simulink model "HMC"  (R2026a)
settings: Solver=ode1  StopTime=inf  FixedStep=0.0001
PreLoadFcn:
  | %load('C:\Users\bme_master\Desktop\mot\mot_6_deneme.mat')
  | 
  | 
  | %load('C:\Users\bme_master\Desktop\mot\PRE_G''s.mat')
PostLoadFcn:
  | , if any(exist('dsrtsu_mdlpostloadfcn', 'file') ~= 0), dsrtsu_mdlpostloadfcn('Execute', bdroot); end,
InitFcn:
  | %motor_control_init_m
  | %clear all
  | %close all
  | %clc
  | b=1e-8
  | StepSize = 1e-4;
  | N=1e-17;
  | 
  | VLV_0 =0;%120; %120
  | VA_0 = 0;%300; %300
  | VRV_0 = 0;%130;
  | VP_0 = 0;%500;
  | VLA_0 = 0;%20;
  | VV_0=5000;
  | VRA_0=0;
  | 
  | 
  | QLV_0 = 0;
  | QLA_0 = 0;
  | QP_0 = 0;
  | 
  | bh = 0;
  | th =0;
  | 
  | X_0 = [VLV_0 VA_0 VV_0 VP_0  VLA_0  VRA_0 VRV_0];
  | 
  | 
  | V0 = 10;
  | 
  | K1=.0004;%0.0001
  | K2=0.0009;%0.0009
  | KA=1;%1
  | C1=0.000000003;%0.0000003
  | lambda=6000;%3000
  | X_00 = [VLV_0 VA_0 VV_0 VRV_0];
  | 
  | r2 = 0.05/2;
  | A2 = pi*r2^2;
  | h2 = 0.63;
  | V2 = A2*h2;
  | 
  | 
  | r3 = 0.05/2;
  | A3 = pi*r3^2;
  | h3 = 0.63;
  | V3 = A3*h3;
  | 
  | 
  | rho = 997;
  | gg = 9.81;
  | %
  | init_min=0;
  | init_max=0;
  | %
  | PWM_Period =  StepSize;
  | PWM_Period_g1 = PWM_Period;
  | PWM_Period_g2 =PWM_Period;
  | PWM_Period_g3 = PWM_Period;
  | PWM_Period_g4 = PWM_Period;
  | PWM_Period_g5 = PWM_Period;
  | PWM_Period_P2_escape = PWM_Period;
  | PWM_Period_P3_escape = PWM_Period;
  | filter_c=100;
  | dt = StepSize;
  | dt_k = dt;
  | rho_g=1.537408456055604
  | Pvac = 0;
  | P1refmmHg = 1600;
  | P2refmmHg = 30;
  | 
  | 
  | P2_ref_freq = 1;
  | P2_ref_bias = 50;
  | P2_ref_amp = 0;
  | P2_ref_shift = 0;
  | Kp = 1;
  | Ki =1;
  | Kd=1;
  | 
  | 
  | P3_ref_freq = 1;
  | P3_ref_bias = 30;
  | P3_ref_amp = 0;
  | P3_ref_shift = 0;
  | 
  | Q_Sys_std = 1;
  | R_Meas_std = 1;
  | kalmanP_in= [133.32*[100 1 10 10 1]]';
  | kalmanQ_in = [1e-3 1e-3]';
  | y_kalman_ini = [133.32*[100 1 10 10 1] 1e-3 1e-3 1e-3]';
  | P_kalman_ini = R_Meas_std^2*eye(8);
  | %P_kalman_ini = R_Meas_std^2*eye(8);
  | %P_kalman_in1 = R_Meas_std^2*eye(8);
  | 
  | 
  | w_gp_0 = 1e-3;
  | i_gp_0 = 1e-3;
  | w_vad_0 = 1e-3;
  | i_vad_0 = 1e-3;
  | 
  | 
  | 
  | 
  | 
  | % e_min = 0.075;
  | % %e_max = 3;
  | % e_max_ill = 1.5; PA_0 = 85;
  | % tau_RA = 1.8;  tau_RV = 3;% 2.3762;
  | % V_total = 5500; V0_la = 70; V0_lv = 120; V0 = 10;
  | % RA = 1.2; Ra = 0.0005;
  | % Rm = 0.0003; Rv = 0.005;
  | % R = [RA Ra Rm Rv];
  | % g = [1/RA 1/Ra 1/Rm 1/Rv];
  | %
  | % CA = tau_RA/RA; CV = tau_RV/Rv;
  | %
  | % V0_aortic = PA_0*CA;
  | % PLV_0 = (V0_lv - V0)*e_min;
  | % CLA = V0_la/PLV_0;
  | % C = [CA CV CLA];
  | % e = [1/CA 1/CV 1/CLA];
  | %
  | % V0_venous = V_total - (V0_aortic + V0_la + V0_lv);
  | % PLA_0 = PLV_0;
  | % PV_0 = V0_venous/CV;
  | 
  | 
  | 
  | 
  | 
  | 
  | 
  | 
  | % stepsize = 1e-4;
  | 
  | % SS=1;
  | 
  | 
  | 
  | 
  | 
  | %global RFa RFp
  | %RFa = 1;
  | %RFmv = 1;
  | 
  | 
  | 
  | 
  | 
  | %L_AV =  0.000232;
  | %L_mv =  0.0001;
  | %L_P =  0.000128;
  | a=0;
  | 
  | 
  | 
  | 
  | 
  | %L= [L_mv];
  | 
  | 
  | 
  | 
  | 
  | % gLV =42;%25;
  | % gA = 0.9225;%0.75;  %0.8;%0.725; %1.11;
  | % gV = 70;%10000;
  | % gRV =210;
  | % gP =5;%15 %10;
  | % gLA = 1000; %1000;
  | %
  | %
  | % G = [gLV gA gV gRV gP gLA];
  | %
  | %
  | % eA =0.5225;%0.725;%1; %0.925;%0.83; %0.65;%0.95;
  | % eV =0.002425;%0.00245;%0.00125;
  | % eP =0.1; %0.01%0.1;
  | % eLA =0.1025;%0.1105%0.1175;%0.15; % 0.15;
  | %
  | %
  | % E = [eA eV eP eLA];
  | %
  | %
  | % ZZ = 0.75;
  | % PP = 0.95;
  | %
  | % V_T = 5000;
  | % VLV_0 =105;%120; %120
  | % VA_0 = 160;%300; %300
  | % VRV_0 = 110;%130;
  | % VP_0 = 200;%500;
  | % VLA_0 = 105;%20;
  | % VV_0=0;
  | % QLV_0 = 0;
  | % QLA_0 = 0;
  | % QP_0 = 0;
  | %
  | % X_0 = [VLV_0 VA_0 VRV_0 VP_0 VLA_0];
  | % %BF_0 = [0 0 0];
  | %
  | %
  | % V0 = 10;
  | 
  | 
  | %Delay = 0.85;
  | 
  | 
  | 
  | 
  | 
  | %%CVS PARAMETERS NEW
  | 
  | 
  | stepsize = 1e-4;
  | 
  | 
  | SS=0.8;
undefined symbols (not defined in the file or in its folder): Continuous, DiscIntNeverNeededParam, Time
libraries: powerlib_meascontrol x19, simulink x15, rti1202lib_adc_class1 x11, cstblocks x10, rti1202lib_dio_class1 x8, dspstat3 x3, rti1202lib_dac_class1 x1, dspswit3 x1, ctrlSharedLib x1, slpidlib x1, dsparch4 x1
(part 1 of 5)
Description:
  | Standard RTI1202 template.
  | Supported MATLAB version:  R2019a.
settings Model: Tag=RTI1202  DSRTSU_INTERNAL_RTI_VER=540  DSRTSU_INTERNAL_RTI_TYPE=rti1202  RTICANMMDATA=struct('GeneralSetupData',struct('modelroot','C:\Users\bme_master\Desktop\dSpaceEncoder','generalsettings',struct('filesettings',struct('destfolder',struct('Name','RTICANMM_FILES','Check',1),'buildfolder',struct('Name','.','Check',1),'AbsDestfolder',struct('Name','C:\Users\bme_master\Desktop\dSpaceEncoder\RTICANMM_FILES'),'AbsBuildfolder',struct('Name','C:\Users\bme_master\Desktop\dSpaceEncoder'))),'options',struct('addpaths',1,'rmpaths',1,'addtrcexclusion',logical(1),'cannavigator',struct('checkmonitoring',0),'show_usrtrc',0,'use_usrtrc',0),'advanced',struct('options',ones(1,100)),'MPSetup',{{}},'RTI',struct('Type','RTI1202','Ver','7.12','Date','02-May-2019'),'modelname','HMC','block','HMC'))  DSRTSU_INTERNAL_RTIFPGA=130  SimulationMode=accelerator  Creator=bme_master  LastModifiedBy=ehd
settings OptimizationCC: OptimizeBlockIOStorage=off  BufferReuse=off  GlobalBufferReuse=off  ExpressionFolding=off  LocalBlockOutputs=off  OptimizeDataStoreBuffers=off  BusAssignmentInplaceUpdate=off
settings HardwareCC: ProdLargestAtomicInteger=Integer  ProdEndianess=BigEndian  ProdHWDeviceType=Custom Processor->Custom  TargetIntDivRoundTo=Zero  TargetEndianess=BigEndian  TargetHWDeviceType=Custom Processor->Custom
settings RTWCC: SystemTargetFile=rti1202.tlc  MakeCommand=make_rti  TemplateMakefile=rti1202.tmf  Description=dSPACE DS1202 Hardware Platform
settings STFCustomTargetCC: SystemTargetFile=rti1202.tlc  MultiwordLength=2048.0  ParMdlRefBuildCompliant=on  GRTInterface=off  InitialSimState=RUN  ExecutionMode=real-time  ExecutionModeNonUI=RTSIM  TaskModeNonUI=LOW_JITTER  TaskMode=Low jitter, low latency tasks  AssertionMode=OFF  TimeScaleFactorNonUI=OPTION_DISABLED  TimeScaleFactor=1.0  EnableRealTimeTesting=on  EnableRealTimeTestingNonUI=ON  LoadAfterBuild=off  CCompilerOptimizationOptsPopup_=Default  CCompilerOptimizationOptsNonUI=USE_DEFAULT  AllowReservedHostServiceNums=off  BoardName=ds1202  RTICfgSetVer=540.0  LoadToFlash=off  TRCGenerateLabels=off  LoadApplNonUI=OFF  PlatformSelectionPopup=Platform Name  TRCGenerateVirtualBlocks=off  BoardNameNonUI=ds1202  NetworkClientNonUI=OPTION_DISABLED  TRCOnlyGlobals=off  TRCGenerateStates=off  TRCGenerateDerivatives=off  TRCGenerateParamValues=off  TRCIsOmitVdOn=off
settings GRTTargetCC: CompOptLevelCompliant=off  ConcurrentExecutionCompliant=off  CombineOutputUpdateFcns=off  MatFileLogging=off  CPPClassGenCompliant=off
settings ConfigComp: CovMetricSettings=dswe
settings SimscapeCC: SimscapeLogType=none  SimscapeNominalValues="[{\"value\":\"1\",\"unit\":\"A\"},{\"value\":\"1\",\"unit\":\"bar\"},{\"value\":\"1\",\"unit\":\"cm^2\"},{\"value\":\"1\",\"unit\":\"cm^3/s\"},{\"value\":\"1\",\"unit\":\"kJ/kg\"},{\"value\":\"1\",\"unit\":\"kW\"},{\"value\":\"1\",\"unit\":\"l\"},{\"value\":\"1\",\"unit\":\"N\"},{\"value\":\"1\",\"unit\":\"N*m\"},{\"value\":\"1\",\"unit\":\"V\"}]"  SimscapeLogDecimation=1  SimscapeLogDataHistory=5000

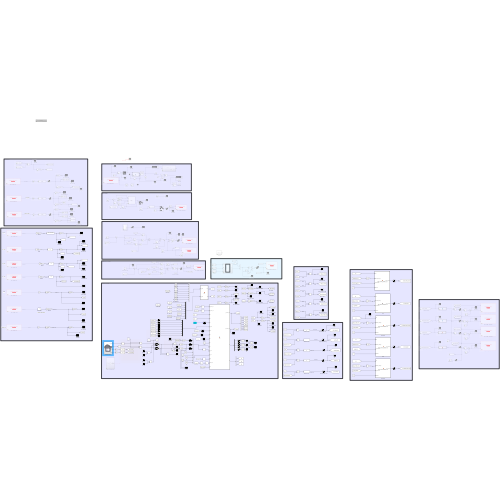
[thumbnail: Simulink's stored preview of the top-level diagram]
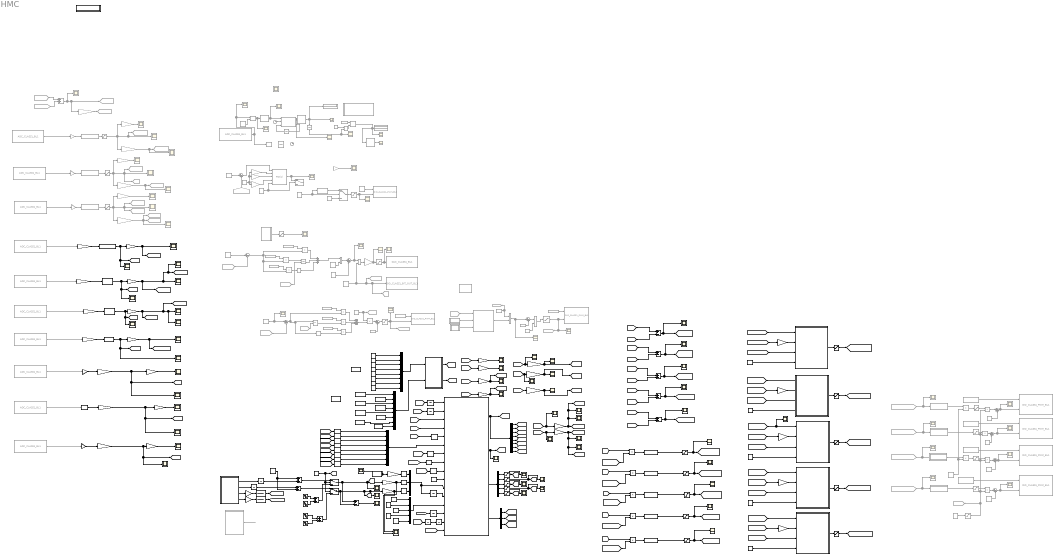
== system HMC ==
  note: ITM Controller
  note: Valve PWM
  note: Flow Sensors
  note: LV_total
  note: DTM LVAD contoller
  note: Ao_pne
  note: Small Pump Controller
  note: GP CONTROLLER
  note: -1 to 0 Bar Conversion
  note: Ao_total
  note: Between Tanks
  note: Comp
  note: Air Flows
  note: Valve Currents
  note: LV_pne
  note: Pressure Differences
  note: Pump Out
  note: Lyapunov controller
  note: Reduction_tank
  ADC_CLASS1_BL1 : rti1202lib_adc_class1/ADC_CLASS1_BL1  Commented=on  DSProperties=struct('RTI',struct('Version',uint32(1),'BlockType',struct('isSLSource',uint8(1),'isSLSink',uint8(1),'isHWSource',uint8(0),'isHWSink',uint8(1),'isSetup',uint8(0),'isInline',uint8(1),'isNonInline',uint8(0),'isInterrupt',uint8(0),'isChannelwise',uint8(1)),'IOBoardType',{{'DS120X','STD','ADCC1'}},'UnitType','ADC','Identifier','ADC','DialogType','ML','BlockSet','NONE','SlaveProcessor','NONE'))  RTIBlockInterface=struct('InputPortsActive',0,'InputPortsWidth',int32(1),'InputPortsDataType',{{'SS_BOOLEAN'}},'InputPortsName',{{'Continue'}},'OutputPortsActive',[1 0],'OutputPortsWidth',int32([1 1]),'OutputPortsDataType',{{'SS_DOUBLE','SS_INT16'}},'OutputPortsName',{{'ADC','Status'}},'DialogFcn','rti120xstdadcc1adcgui','SampleTime',{{-1}},'InitLevel',3,'IconTransparency','on','BlockDisplay',{{['ADC CL1\nChannel: 10'],'center'}},'BlockName',struct('Token',{{'ADC_CLASS1_BL1'}}))  RTIBlockParameters=struct('ReadMode',{{1,'OFF',[1 2]}},'ChannelNo',{{10,'OFF',[]}},'ConversionMode',{{1,'OFF',[1 2]}},'TriggerSource',{{1,'OFF',[1 2]}},'TriggerLineIn',{{1,'OFF',[1 16]}},'SampleMode',{{1,'OFF',[1 2]}},'BurstTriggerSource',{{1,'OFF',[1 2]}},'BurstTriggerLine',{{1,'OFF',[1 16]}},'ConvTriggerSource',{{3,'OFF',[1 3]}},'ConvTriggerLine',{{1,'OFF',[1 16]}},'ConvPeriod',{{'100e-6','OFF',[1e-6 1.34]}},'ConvPeriodCheck',{{0,'OFF',[]}},'BurstSize',{{'10','OFF',[]}},'BurstSizeCheck',{{0,'OFF',[]}},'DataSetOffset',{{'0','OFF',[]}},'DataSetOffsetCheck',{{0,'OFF',[]}},'DataSetLength',{{'1','OFF',[]}},'DataSetLengthCheck',{{0,'OFF',[]}},'EnableTriggerEvent',{{0,'OFF',[0 1]}},'TriggerMode',{{2,'OFF',[1 3]}},'TriggerLineOut',{{1,'OFF',[1 16]}},'ADCSWStartEnable',{{0,'OFF',[0 1]}},'SampleTime',{{'-1','OFF',[-1 inf]}},'SampleTimeCheck',{{1,'OFF',[]}},'StatusPortEnable',{{0,'OFF',[0 1]}},'TLCFileName',{{'rti120xadc_c1_adc','OFF',[]}})  RTISFcnParameters=struct('ReadMode','int16','ChannelNo','int16','ConversionMode','int16','TriggerSource','int16','TriggerLineIn','int16','SampleMode','int16','BurstTriggerSource','int16','BurstTriggerLine','int16','ConvTriggerSource','int16','ConvTriggerLine','int16','ConvPeriod','double','BurstSize','int16','DataSetOffset','int16','DataSetLength','int16','EnableTriggerEvent','int16','TriggerMode','int16','TriggerLineOut','int16','ADCSWStartEnable','int16','SampleTime','double','StatusPortEnable','int16','TLCFileName','char')  RTIBlockParaDefault=struct('ReadMode',1,'ChannelNo',1,'ConversionMode',1,'TriggerSource',1,'TriggerLineIn',1,'SampleMode',1,'BurstTriggerSource',1,'BurstTriggerLine',1,'ConvTriggerSource',3,'ConvTriggerLine',1,'ConvPeriod',0.0001,'ConvPeriodCheck',0,'BurstSize',10,'BurstSizeCheck',0,'DataSetOffset',0,'DataSetOffsetCheck',0,'DataSetLength',1,'DataSetLengthCheck',0,'EnableTriggerEvent',0,'TriggerMode',2,'TriggerLineOut',1,'ADCSWStartEnable',0,'SampleTime',-1,'SampleTimeCheck',1,'StatusPortEnable',0,'TLCFileName','rti120xadc_c1_adc')
  ADC_CLASS1_BL11 : rti1202lib_adc_class1/ADC_CLASS1_BL1  Commented=on  DSProperties=struct('RTI',struct('Version',uint32(1),'BlockType',struct('isSLSource',uint8(1),'isSLSink',uint8(1),'isHWSource',uint8(0),'isHWSink',uint8(1),'isSetup',uint8(0),'isInline',uint8(1),'isNonInline',uint8(0),'isInterrupt',uint8(0),'isChannelwise',uint8(1)),'IOBoardType',{{'DS120X','STD','ADCC1'}},'UnitType','ADC','Identifier','ADC','DialogType','ML','BlockSet','NONE','SlaveProcessor','NONE'))  RTIBlockInterface=struct('InputPortsActive',0,'InputPortsWidth',int32(1),'InputPortsDataType',{{'SS_BOOLEAN'}},'InputPortsName',{{'Continue'}},'OutputPortsActive',[1 0],'OutputPortsWidth',int32([1 1]),'OutputPortsDataType',{{'SS_DOUBLE','SS_INT16'}},'OutputPortsName',{{'ADC','Status'}},'DialogFcn','rti120xstdadcc1adcgui','SampleTime',{{-1}},'InitLevel',3,'IconTransparency','on','BlockDisplay',{{['ADC CL1\nChannel: 4'],'center'}},'BlockName',struct('Token',{{'ADC_CLASS1_BL1'}}))  RTIBlockParameters=struct('ReadMode',{{1,'OFF',[1 2]}},'ChannelNo',{{4,'OFF',[]}},'ConversionMode',{{1,'OFF',[1 2]}},'TriggerSource',{{1,'OFF',[1 2]}},'TriggerLineIn',{{1,'OFF',[1 16]}},'SampleMode',{{1,'OFF',[1 2]}},'BurstTriggerSource',{{1,'OFF',[1 2]}},'BurstTriggerLine',{{1,'OFF',[1 16]}},'ConvTriggerSource',{{3,'OFF',[1 3]}},'ConvTriggerLine',{{1,'OFF',[1 16]}},'ConvPeriod',{{'100e-6','OFF',[1e-6 1.34]}},'ConvPeriodCheck',{{0,'OFF',[]}},'BurstSize',{{'10','OFF',[]}},'BurstSizeCheck',{{0,'OFF',[]}},'DataSetOffset',{{'0','OFF',[]}},'DataSetOffsetCheck',{{0,'OFF',[]}},'DataSetLength',{{'1','OFF',[]}},'DataSetLengthCheck',{{0,'OFF',[]}},'EnableTriggerEvent',{{0,'OFF',[0 1]}},'TriggerMode',{{2,'OFF',[1 3]}},'TriggerLineOut',{{1,'OFF',[1 16]}},'ADCSWStartEnable',{{0,'OFF',[0 1]}},'SampleTime',{{'-1','OFF',[-1 inf]}},'SampleTimeCheck',{{1,'OFF',[]}},'StatusPortEnable',{{0,'OFF',[0 1]}},'TLCFileName',{{'rti120xadc_c1_adc','OFF',[]}})  RTISFcnParameters=struct('ReadMode','int16','ChannelNo','int16','ConversionMode','int16','TriggerSource','int16','TriggerLineIn','int16','SampleMode','int16','BurstTriggerSource','int16','BurstTriggerLine','int16','ConvTriggerSource','int16','ConvTriggerLine','int16','ConvPeriod','double','BurstSize','int16','DataSetOffset','int16','DataSetLength','int16','EnableTriggerEvent','int16','TriggerMode','int16','TriggerLineOut','int16','ADCSWStartEnable','int16','SampleTime','double','StatusPortEnable','int16','TLCFileName','char')  RTIBlockParaDefault=struct('ReadMode',1,'ChannelNo',1,'ConversionMode',1,'TriggerSource',1,'TriggerLineIn',1,'SampleMode',1,'BurstTriggerSource',1,'BurstTriggerLine',1,'ConvTriggerSource',3,'ConvTriggerLine',1,'ConvPeriod',0.0001,'ConvPeriodCheck',0,'BurstSize',10,'BurstSizeCheck',0,'DataSetOffset',0,'DataSetOffsetCheck',0,'DataSetLength',1,'DataSetLengthCheck',0,'EnableTriggerEvent',0,'TriggerMode',2,'TriggerLineOut',1,'ADCSWStartEnable',0,'SampleTime',-1,'SampleTimeCheck',1,'StatusPortEnable',0,'TLCFileName','rti120xadc_c1_adc')
  ADC_CLASS1_BL12 : rti1202lib_adc_class1/ADC_CLASS1_BL1  Commented=on  DSProperties=struct('RTI',struct('Version',uint32(1),'BlockType',struct('isSLSource',uint8(1),'isSLSink',uint8(1),'isHWSource',uint8(0),'isHWSink',uint8(1),'isSetup',uint8(0),'isInline',uint8(1),'isNonInline',uint8(0),'isInterrupt',uint8(0),'isChannelwise',uint8(1)),'IOBoardType',{{'DS120X','STD','ADCC1'}},'UnitType','ADC','Identifier','ADC','DialogType','ML','BlockSet','NONE','SlaveProcessor','NONE'))  RTIBlockInterface=struct('InputPortsActive',0,'InputPortsWidth',int32(1),'InputPortsDataType',{{'SS_BOOLEAN'}},'InputPortsName',{{'Continue'}},'OutputPortsActive',[1 0],'OutputPortsWidth',int32([1 1]),'OutputPortsDataType',{{'SS_DOUBLE','SS_INT16'}},'OutputPortsName',{{'ADC','Status'}},'DialogFcn','rti120xstdadcc1adcgui','SampleTime',{{-1}},'InitLevel',3,'IconTransparency','on','BlockDisplay',{{['ADC CL1\nChannel: 6'],'center'}},'BlockName',struct('Token',{{'ADC_CLASS1_BL1'}}))  RTIBlockParameters=struct('ReadMode',{{1,'OFF',[1 2]}},'ChannelNo',{{6,'OFF',[]}},'ConversionMode',{{1,'OFF',[1 2]}},'TriggerSource',{{1,'OFF',[1 2]}},'TriggerLineIn',{{1,'OFF',[1 16]}},'SampleMode',{{1,'OFF',[1 2]}},'BurstTriggerSource',{{1,'OFF',[1 2]}},'BurstTriggerLine',{{1,'OFF',[1 16]}},'ConvTriggerSource',{{3,'OFF',[1 3]}},'ConvTriggerLine',{{1,'OFF',[1 16]}},'ConvPeriod',{{'100e-6','OFF',[1e-6 1.34]}},'ConvPeriodCheck',{{0,'OFF',[]}},'BurstSize',{{'10','OFF',[]}},'BurstSizeCheck',{{0,'OFF',[]}},'DataSetOffset',{{'0','OFF',[]}},'DataSetOffsetCheck',{{0,'OFF',[]}},'DataSetLength',{{'1','OFF',[]}},'DataSetLengthCheck',{{0,'OFF',[]}},'EnableTriggerEvent',{{0,'OFF',[0 1]}},'TriggerMode',{{2,'OFF',[1 3]}},'TriggerLineOut',{{1,'OFF',[1 16]}},'ADCSWStartEnable',{{0,'OFF',[0 1]}},'SampleTime',{{'-1','OFF',[-1 inf]}},'SampleTimeCheck',{{1,'OFF',[]}},'StatusPortEnable',{{0,'OFF',[0 1]}},'TLCFileName',{{'rti120xadc_c1_adc','OFF',[]}})  RTISFcnParameters=struct('ReadMode','int16','ChannelNo','int16','ConversionMode','int16','TriggerSource','int16','TriggerLineIn','int16','SampleMode','int16','BurstTriggerSource','int16','BurstTriggerLine','int16','ConvTriggerSource','int16','ConvTriggerLine','int16','ConvPeriod','double','BurstSize','int16','DataSetOffset','int16','DataSetLength','int16','EnableTriggerEvent','int16','TriggerMode','int16','TriggerLineOut','int16','ADCSWStartEnable','int16','SampleTime','double','StatusPortEnable','int16','TLCFileName','char')  RTIBlockParaDefault=struct('ReadMode',1,'ChannelNo',1,'ConversionMode',1,'TriggerSource',1,'TriggerLineIn',1,'SampleMode',1,'BurstTriggerSource',1,'BurstTriggerLine',1,'ConvTriggerSource',3,'ConvTriggerLine',1,'ConvPeriod',0.0001,'ConvPeriodCheck',0,'BurstSize',10,'BurstSizeCheck',0,'DataSetOffset',0,'DataSetOffsetCheck',0,'DataSetLength',1,'DataSetLengthCheck',0,'EnableTriggerEvent',0,'TriggerMode',2,'TriggerLineOut',1,'ADCSWStartEnable',0,'SampleTime',-1,'SampleTimeCheck',1,'StatusPortEnable',0,'TLCFileName','rti120xadc_c1_adc')
  ADC_CLASS1_BL13 : rti1202lib_adc_class1/ADC_CLASS1_BL1  Commented=on  DSProperties=struct('RTI',struct('Version',uint32(1),'BlockType',struct('isSLSource',uint8(1),'isSLSink',uint8(1),'isHWSource',uint8(0),'isHWSink',uint8(1),'isSetup',uint8(0),'isInline',uint8(1),'isNonInline',uint8(0),'isInterrupt',uint8(0),'isChannelwise',uint8(1)),'IOBoardType',{{'DS120X','STD','ADCC1'}},'UnitType','ADC','Identifier','ADC','DialogType','ML','BlockSet','NONE','SlaveProcessor','NONE'))  RTIBlockInterface=struct('InputPortsActive',0,'InputPortsWidth',int32(1),'InputPortsDataType',{{'SS_BOOLEAN'}},'InputPortsName',{{'Continue'}},'OutputPortsActive',[1 0],'OutputPortsWidth',int32([1 1]),'OutputPortsDataType',{{'SS_DOUBLE','SS_INT16'}},'OutputPortsName',{{'ADC','Status'}},'DialogFcn','rti120xstdadcc1adcgui','SampleTime',{{-1}},'InitLevel',3,'IconTransparency','on','BlockDisplay',{{['ADC CL1\nChannel: 11'],'center'}},'BlockName',struct('Token',{{'ADC_CLASS1_BL1'}}))  RTIBlockParameters=struct('ReadMode',{{1,'OFF',[1 2]}},'ChannelNo',{{11,'OFF',[]}},'ConversionMode',{{1,'OFF',[1 2]}},'TriggerSource',{{1,'OFF',[1 2]}},'TriggerLineIn',{{1,'OFF',[1 16]}},'SampleMode',{{1,'OFF',[1 2]}},'BurstTriggerSource',{{1,'OFF',[1 2]}},'BurstTriggerLine',{{1,'OFF',[1 16]}},'ConvTriggerSource',{{3,'OFF',[1 3]}},'ConvTriggerLine',{{1,'OFF',[1 16]}},'ConvPeriod',{{'100e-6','OFF',[1e-6 1.34]}},'ConvPeriodCheck',{{0,'OFF',[]}},'BurstSize',{{'10','OFF',[]}},'BurstSizeCheck',{{0,'OFF',[]}},'DataSetOffset',{{'0','OFF',[]}},'DataSetOffsetCheck',{{0,'OFF',[]}},'DataSetLength',{{'1','OFF',[]}},'DataSetLengthCheck',{{0,'OFF',[]}},'EnableTriggerEvent',{{0,'OFF',[0 1]}},'TriggerMode',{{2,'OFF',[1 3]}},'TriggerLineOut',{{1,'OFF',[1 16]}},'ADCSWStartEnable',{{0,'OFF',[0 1]}},'SampleTime',{{'-1','OFF',[-1 inf]}},'SampleTimeCheck',{{1,'OFF',[]}},'StatusPortEnable',{{0,'OFF',[0 1]}},'TLCFileName',{{'rti120xadc_c1_adc','OFF',[]}})  RTISFcnParameters=struct('ReadMode','int16','ChannelNo','int16','ConversionMode','int16','TriggerSource','int16','TriggerLineIn','int16','SampleMode','int16','BurstTriggerSource','int16','BurstTriggerLine','int16','ConvTriggerSource','int16','ConvTriggerLine','int16','ConvPeriod','double','BurstSize','int16','DataSetOffset','int16','DataSetLength','int16','EnableTriggerEvent','int16','TriggerMode','int16','TriggerLineOut','int16','ADCSWStartEnable','int16','SampleTime','double','StatusPortEnable','int16','TLCFileName','char')  RTIBlockParaDefault=struct('ReadMode',1,'ChannelNo',1,'ConversionMode',1,'TriggerSource',1,'TriggerLineIn',1,'SampleMode',1,'BurstTriggerSource',1,'BurstTriggerLine',1,'ConvTriggerSource',3,'ConvTriggerLine',1,'ConvPeriod',0.0001,'ConvPeriodCheck',0,'BurstSize',10,'BurstSizeCheck',0,'DataSetOffset',0,'DataSetOffsetCheck',0,'DataSetLength',1,'DataSetLengthCheck',0,'EnableTriggerEvent',0,'TriggerMode',2,'TriggerLineOut',1,'ADCSWStartEnable',0,'SampleTime',-1,'SampleTimeCheck',1,'StatusPortEnable',0,'TLCFileName','rti120xadc_c1_adc')
  ADC_CLASS1_BL14 : rti1202lib_adc_class1/ADC_CLASS1_BL1  Commented=on  DSProperties=struct('RTI',struct('Version',uint32(1),'BlockType',struct('isSLSource',uint8(1),'isSLSink',uint8(1),'isHWSource',uint8(0),'isHWSink',uint8(1),'isSetup',uint8(0),'isInline',uint8(1),'isNonInline',uint8(0),'isInterrupt',uint8(0),'isChannelwise',uint8(1)),'IOBoardType',{{'DS120X','STD','ADCC1'}},'UnitType','ADC','Identifier','ADC','DialogType','ML','BlockSet','NONE','SlaveProcessor','NONE'))  RTIBlockInterface=struct('InputPortsActive',0,'InputPortsWidth',int32(1),'InputPortsDataType',{{'SS_BOOLEAN'}},'InputPortsName',{{'Continue'}},'OutputPortsActive',[1 0],'OutputPortsWidth',int32([1 1]),'OutputPortsDataType',{{'SS_DOUBLE','SS_INT16'}},'OutputPortsName',{{'ADC','Status'}},'DialogFcn','rti120xstdadcc1adcgui','SampleTime',{{-1}},'InitLevel',3,'IconTransparency','on','BlockDisplay',{{['ADC CL1\nChannel: 23'],'center'}},'BlockName',struct('Token',{{'ADC_CLASS1_BL1'}}))  RTIBlockParameters=struct('ReadMode',{{1,'OFF',[1 2]}},'ChannelNo',{{23,'OFF',[]}},'ConversionMode',{{1,'OFF',[1 2]}},'TriggerSource',{{1,'OFF',[1 2]}},'TriggerLineIn',{{1,'OFF',[1 16]}},'SampleMode',{{1,'OFF',[1 2]}},'BurstTriggerSource',{{1,'OFF',[1 2]}},'BurstTriggerLine',{{1,'OFF',[1 16]}},'ConvTriggerSource',{{3,'OFF',[1 3]}},'ConvTriggerLine',{{1,'OFF',[1 16]}},'ConvPeriod',{{'100e-6','OFF',[1e-6 1.34]}},'ConvPeriodCheck',{{0,'OFF',[]}},'BurstSize',{{'10','OFF',[]}},'BurstSizeCheck',{{0,'OFF',[]}},'DataSetOffset',{{'0','OFF',[]}},'DataSetOffsetCheck',{{0,'OFF',[]}},'DataSetLength',{{'1','OFF',[]}},'DataSetLengthCheck',{{0,'OFF',[]}},'EnableTriggerEvent',{{0,'OFF',[0 1]}},'TriggerMode',{{2,'OFF',[1 3]}},'TriggerLineOut',{{1,'OFF',[1 16]}},'ADCSWStartEnable',{{0,'OFF',[0 1]}},'SampleTime',{{'-1','OFF',[-1 inf]}},'SampleTimeCheck',{{1,'OFF',[]}},'StatusPortEnable',{{0,'OFF',[0 1]}},'TLCFileName',{{'rti120xadc_c1_adc','OFF',[]}})  RTISFcnParameters=struct('ReadMode','int16','ChannelNo','int16','ConversionMode','int16','TriggerSource','int16','TriggerLineIn','int16','SampleMode','int16','BurstTriggerSource','int16','BurstTriggerLine','int16','ConvTriggerSource','int16','ConvTriggerLine','int16','ConvPeriod','double','BurstSize','int16','DataSetOffset','int16','DataSetLength','int16','EnableTriggerEvent','int16','TriggerMode','int16','TriggerLineOut','int16','ADCSWStartEnable','int16','SampleTime','double','StatusPortEnable','int16','TLCFileName','char')  RTIBlockParaDefault=struct('ReadMode',1,'ChannelNo',1,'ConversionMode',1,'TriggerSource',1,'TriggerLineIn',1,'SampleMode',1,'BurstTriggerSource',1,'BurstTriggerLine',1,'ConvTriggerSource',3,'ConvTriggerLine',1,'ConvPeriod',0.0001,'ConvPeriodCheck',0,'BurstSize',10,'BurstSizeCheck',0,'DataSetOffset',0,'DataSetOffsetCheck',0,'DataSetLength',1,'DataSetLengthCheck',0,'EnableTriggerEvent',0,'TriggerMode',2,'TriggerLineOut',1,'ADCSWStartEnable',0,'SampleTime',-1,'SampleTimeCheck',1,'StatusPortEnable',0,'TLCFileName','rti120xadc_c1_adc')
  ADC_CLASS1_BL2 : rti1202lib_adc_class1/ADC_CLASS1_BL1  Commented=on  DSProperties=struct('RTI',struct('Version',uint32(1),'BlockType',struct('isSLSource',uint8(1),'isSLSink',uint8(1),'isHWSource',uint8(0),'isHWSink',uint8(1),'isSetup',uint8(0),'isInline',uint8(1),'isNonInline',uint8(0),'isInterrupt',uint8(0),'isChannelwise',uint8(1)),'IOBoardType',{{'DS120X','STD','ADCC1'}},'UnitType','ADC','Identifier','ADC','DialogType','ML','BlockSet','NONE','SlaveProcessor','NONE'))  RTIBlockInterface=struct('InputPortsActive',0,'InputPortsWidth',int32(1),'InputPortsDataType',{{'SS_BOOLEAN'}},'InputPortsName',{{'Continue'}},'OutputPortsActive',[1 0],'OutputPortsWidth',int32([1 1]),'OutputPortsDataType',{{'SS_DOUBLE','SS_INT16'}},'OutputPortsName',{{'ADC','Status'}},'DialogFcn','rti120xstdadcc1adcgui','SampleTime',{{-1}},'InitLevel',3,'IconTransparency','on','BlockDisplay',{{['ADC CL1\nChannel: 3'],'center'}},'BlockName',struct('Token',{{'ADC_CLASS1_BL1'}}))  RTIBlockParameters=struct('ReadMode',{{1,'OFF',[1 2]}},'ChannelNo',{{3,'OFF',[]}},'ConversionMode',{{1,'OFF',[1 2]}},'TriggerSource',{{1,'OFF',[1 2]}},'TriggerLineIn',{{1,'OFF',[1 16]}},'SampleMode',{{1,'OFF',[1 2]}},'BurstTriggerSource',{{1,'OFF',[1 2]}},'BurstTriggerLine',{{1,'OFF',[1 16]}},'ConvTriggerSource',{{3,'OFF',[1 3]}},'ConvTriggerLine',{{1,'OFF',[1 16]}},'ConvPeriod',{{'100e-6','OFF',[1e-6 1.34]}},'ConvPeriodCheck',{{0,'OFF',[]}},'BurstSize',{{'10','OFF',[]}},'BurstSizeCheck',{{0,'OFF',[]}},'DataSetOffset',{{'0','OFF',[]}},'DataSetOffsetCheck',{{0,'OFF',[]}},'DataSetLength',{{'1','OFF',[]}},'DataSetLengthCheck',{{0,'OFF',[]}},'EnableTriggerEvent',{{0,'OFF',[0 1]}},'TriggerMode',{{2,'OFF',[1 3]}},'TriggerLineOut',{{1,'OFF',[1 16]}},'ADCSWStartEnable',{{0,'OFF',[0 1]}},'SampleTime',{{'-1','OFF',[-1 inf]}},'SampleTimeCheck',{{1,'OFF',[]}},'StatusPortEnable',{{0,'OFF',[0 1]}},'TLCFileName',{{'rti120xadc_c1_adc','OFF',[]}})  RTISFcnParameters=struct('ReadMode','int16','ChannelNo','int16','ConversionMode','int16','TriggerSource','int16','TriggerLineIn','int16','SampleMode','int16','BurstTriggerSource','int16','BurstTriggerLine','int16','ConvTriggerSource','int16','ConvTriggerLine','int16','ConvPeriod','double','BurstSize','int16','DataSetOffset','int16','DataSetLength','int16','EnableTriggerEvent','int16','TriggerMode','int16','TriggerLineOut','int16','ADCSWStartEnable','int16','SampleTime','double','StatusPortEnable','int16','TLCFileName','char')  RTIBlockParaDefault=struct('ReadMode',1,'ChannelNo',1,'ConversionMode',1,'TriggerSource',1,'TriggerLineIn',1,'SampleMode',1,'BurstTriggerSource',1,'BurstTriggerLine',1,'ConvTriggerSource',3,'ConvTriggerLine',1,'ConvPeriod',0.0001,'ConvPeriodCheck',0,'BurstSize',10,'BurstSizeCheck',0,'DataSetOffset',0,'DataSetOffsetCheck',0,'DataSetLength',1,'DataSetLengthCheck',0,'EnableTriggerEvent',0,'TriggerMode',2,'TriggerLineOut',1,'ADCSWStartEnable',0,'SampleTime',-1,'SampleTimeCheck',1,'StatusPortEnable',0,'TLCFileName','rti120xadc_c1_adc')
  ADC_CLASS1_BL3 : rti1202lib_adc_class1/ADC_CLASS1_BL1  Commented=on  DSProperties=struct('RTI',struct('Version',uint32(1),'BlockType',struct('isSLSource',uint8(1),'isSLSink',uint8(1),'isHWSource',uint8(0),'isHWSink',uint8(1),'isSetup',uint8(0),'isInline',uint8(1),'isNonInline',uint8(0),'isInterrupt',uint8(0),'isChannelwise',uint8(1)),'IOBoardType',{{'DS120X','STD','ADCC1'}},'UnitType','ADC','Identifier','ADC','DialogType','ML','BlockSet','NONE','SlaveProcessor','NONE'))  RTIBlockInterface=struct('InputPortsActive',0,'InputPortsWidth',int32(1),'InputPortsDataType',{{'SS_BOOLEAN'}},'InputPortsName',{{'Continue'}},'OutputPortsActive',[1 0],'OutputPortsWidth',int32([1 1]),'OutputPortsDataType',{{'SS_DOUBLE','SS_INT16'}},'OutputPortsName',{{'ADC','Status'}},'DialogFcn','rti120xstdadcc1adcgui','SampleTime',{{-1}},'InitLevel',3,'IconTransparency','on','BlockDisplay',{{['ADC CL1\nChannel: 2'],'center'}},'BlockName',struct('Token',{{'ADC_CLASS1_BL1'}}))  RTIBlockParameters=struct('ReadMode',{{1,'OFF',[1 2]}},'ChannelNo',{{2,'OFF',[]}},'ConversionMode',{{1,'OFF',[1 2]}},'TriggerSource',{{1,'OFF',[1 2]}},'TriggerLineIn',{{1,'OFF',[1 16]}},'SampleMode',{{1,'OFF',[1 2]}},'BurstTriggerSource',{{1,'OFF',[1 2]}},'BurstTriggerLine',{{1,'OFF',[1 16]}},'ConvTriggerSource',{{3,'OFF',[1 3]}},'ConvTriggerLine',{{1,'OFF',[1 16]}},'ConvPeriod',{{'100e-6','OFF',[1e-6 1.34]}},'ConvPeriodCheck',{{0,'OFF',[]}},'BurstSize',{{'10','OFF',[]}},'BurstSizeCheck',{{0,'OFF',[]}},'DataSetOffset',{{'0','OFF',[]}},'DataSetOffsetCheck',{{0,'OFF',[]}},'DataSetLength',{{'1','OFF',[]}},'DataSetLengthCheck',{{0,'OFF',[]}},'EnableTriggerEvent',{{0,'OFF',[0 1]}},'TriggerMode',{{2,'OFF',[1 3]}},'TriggerLineOut',{{1,'OFF',[1 16]}},'ADCSWStartEnable',{{0,'OFF',[0 1]}},'SampleTime',{{'-1','OFF',[-1 inf]}},'SampleTimeCheck',{{1,'OFF',[]}},'StatusPortEnable',{{0,'OFF',[0 1]}},'TLCFileName',{{'rti120xadc_c1_adc','OFF',[]}})  RTISFcnParameters=struct('ReadMode','int16','ChannelNo','int16','ConversionMode','int16','TriggerSource','int16','TriggerLineIn','int16','SampleMode','int16','BurstTriggerSource','int16','BurstTriggerLine','int16','ConvTriggerSource','int16','ConvTriggerLine','int16','ConvPeriod','double','BurstSize','int16','DataSetOffset','int16','DataSetLength','int16','EnableTriggerEvent','int16','TriggerMode','int16','TriggerLineOut','int16','ADCSWStartEnable','int16','SampleTime','double','StatusPortEnable','int16','TLCFileName','char')  RTIBlockParaDefault=struct('ReadMode',1,'ChannelNo',1,'ConversionMode',1,'TriggerSource',1,'TriggerLineIn',1,'SampleMode',1,'BurstTriggerSource',1,'BurstTriggerLine',1,'ConvTriggerSource',3,'ConvTriggerLine',1,'ConvPeriod',0.0001,'ConvPeriodCheck',0,'BurstSize',10,'BurstSizeCheck',0,'DataSetOffset',0,'DataSetOffsetCheck',0,'DataSetLength',1,'DataSetLengthCheck',0,'EnableTriggerEvent',0,'TriggerMode',2,'TriggerLineOut',1,'ADCSWStartEnable',0,'SampleTime',-1,'SampleTimeCheck',1,'StatusPortEnable',0,'TLCFileName','rti120xadc_c1_adc')
  ADC_CLASS1_BL4 : rti1202lib_adc_class1/ADC_CLASS1_BL1  Commented=on  DSProperties=struct('RTI',struct('Version',uint32(1),'BlockType',struct('isSLSource',uint8(1),'isSLSink',uint8(1),'isHWSource',uint8(0),'isHWSink',uint8(1),'isSetup',uint8(0),'isInline',uint8(1),'isNonInline',uint8(0),'isInterrupt',uint8(0),'isChannelwise',uint8(1)),'IOBoardType',{{'DS120X','STD','ADCC1'}},'UnitType','ADC','Identifier','ADC','DialogType','ML','BlockSet','NONE','SlaveProcessor','NONE'))  RTIBlockInterface=struct('InputPortsActive',0,'InputPortsWidth',int32(1),'InputPortsDataType',{{'SS_BOOLEAN'}},'InputPortsName',{{'Continue'}},'OutputPortsActive',[1 0],'OutputPortsWidth',int32([1 1]),'OutputPortsDataType',{{'SS_DOUBLE','SS_INT16'}},'OutputPortsName',{{'ADC','Status'}},'DialogFcn','rti120xstdadcc1adcgui','SampleTime',{{-1}},'InitLevel',3,'IconTransparency','on','BlockDisplay',{{['ADC CL1\nChannel: 9'],'center'}},'BlockName',struct('Token',{{'ADC_CLASS1_BL1'}}))  RTIBlockParameters=struct('ReadMode',{{1,'OFF',[1 2]}},'ChannelNo',{{9,'OFF',[]}},'ConversionMode',{{1,'OFF',[1 2]}},'TriggerSource',{{1,'OFF',[1 2]}},'TriggerLineIn',{{1,'OFF',[1 16]}},'SampleMode',{{1,'OFF',[1 2]}},'BurstTriggerSource',{{1,'OFF',[1 2]}},'BurstTriggerLine',{{1,'OFF',[1 16]}},'ConvTriggerSource',{{3,'OFF',[1 3]}},'ConvTriggerLine',{{1,'OFF',[1 16]}},'ConvPeriod',{{'100e-6','OFF',[1e-6 1.34]}},'ConvPeriodCheck',{{0,'OFF',[]}},'BurstSize',{{'10','OFF',[]}},'BurstSizeCheck',{{0,'OFF',[]}},'DataSetOffset',{{'0','OFF',[]}},'DataSetOffsetCheck',{{0,'OFF',[]}},'DataSetLength',{{'1','OFF',[]}},'DataSetLengthCheck',{{0,'OFF',[]}},'EnableTriggerEvent',{{0,'OFF',[0 1]}},'TriggerMode',{{2,'OFF',[1 3]}},'TriggerLineOut',{{1,'OFF',[1 16]}},'ADCSWStartEnable',{{0,'OFF',[0 1]}},'SampleTime',{{'-1','OFF',[-1 inf]}},'SampleTimeCheck',{{1,'OFF',[]}},'StatusPortEnable',{{0,'OFF',[0 1]}},'TLCFileName',{{'rti120xadc_c1_adc','OFF',[]}})  RTISFcnParameters=struct('ReadMode','int16','ChannelNo','int16','ConversionMode','int16','TriggerSource','int16','TriggerLineIn','int16','SampleMode','int16','BurstTriggerSource','int16','BurstTriggerLine','int16','ConvTriggerSource','int16','ConvTriggerLine','int16','ConvPeriod','double','BurstSize','int16','DataSetOffset','int16','DataSetLength','int16','EnableTriggerEvent','int16','TriggerMode','int16','TriggerLineOut','int16','ADCSWStartEnable','int16','SampleTime','double','StatusPortEnable','int16','TLCFileName','char')  RTIBlockParaDefault=struct('ReadMode',1,'ChannelNo',1,'ConversionMode',1,'TriggerSource',1,'TriggerLineIn',1,'SampleMode',1,'BurstTriggerSource',1,'BurstTriggerLine',1,'ConvTriggerSource',3,'ConvTriggerLine',1,'ConvPeriod',0.0001,'ConvPeriodCheck',0,'BurstSize',10,'BurstSizeCheck',0,'DataSetOffset',0,'DataSetOffsetCheck',0,'DataSetLength',1,'DataSetLengthCheck',0,'EnableTriggerEvent',0,'TriggerMode',2,'TriggerLineOut',1,'ADCSWStartEnable',0,'SampleTime',-1,'SampleTimeCheck',1,'StatusPortEnable',0,'TLCFileName','rti120xadc_c1_adc')
  ADC_CLASS1_BL5 : rti1202lib_adc_class1/ADC_CLASS1_BL1  Commented=on  DSProperties=struct('RTI',struct('Version',uint32(1),'BlockType',struct('isSLSource',uint8(1),'isSLSink',uint8(1),'isHWSource',uint8(0),'isHWSink',uint8(1),'isSetup',uint8(0),'isInline',uint8(1),'isNonInline',uint8(0),'isInterrupt',uint8(0),'isChannelwise',uint8(1)),'IOBoardType',{{'DS120X','STD','ADCC1'}},'UnitType','ADC','Identifier','ADC','DialogType','ML','BlockSet','NONE','SlaveProcessor','NONE'))  RTIBlockInterface=struct('InputPortsActive',0,'InputPortsWidth',int32(1),'InputPortsDataType',{{'SS_BOOLEAN'}},'InputPortsName',{{'Continue'}},'OutputPortsActive',[1 0],'OutputPortsWidth',int32([1 1]),'OutputPortsDataType',{{'SS_DOUBLE','SS_INT16'}},'OutputPortsName',{{'ADC','Status'}},'DialogFcn','rti120xstdadcc1adcgui','SampleTime',{{-1}},'InitLevel',3,'IconTransparency','on','BlockDisplay',{{['ADC CL1\nChannel: 13'],'center'}},'BlockName',struct('Token',{{'ADC_CLASS1_BL1'}}))  RTIBlockParameters=struct('ReadMode',{{1,'OFF',[1 2]}},'ChannelNo',{{13,'OFF',[]}},'ConversionMode',{{1,'OFF',[1 2]}},'TriggerSource',{{1,'OFF',[1 2]}},'TriggerLineIn',{{1,'OFF',[1 16]}},'SampleMode',{{1,'OFF',[1 2]}},'BurstTriggerSource',{{1,'OFF',[1 2]}},'BurstTriggerLine',{{1,'OFF',[1 16]}},'ConvTriggerSource',{{3,'OFF',[1 3]}},'ConvTriggerLine',{{1,'OFF',[1 16]}},'ConvPeriod',{{'100e-6','OFF',[1e-6 1.34]}},'ConvPeriodCheck',{{0,'OFF',[]}},'BurstSize',{{'10','OFF',[]}},'BurstSizeCheck',{{0,'OFF',[]}},'DataSetOffset',{{'0','OFF',[]}},'DataSetOffsetCheck',{{0,'OFF',[]}},'DataSetLength',{{'1','OFF',[]}},'DataSetLengthCheck',{{0,'OFF',[]}},'EnableTriggerEvent',{{0,'OFF',[0 1]}},'TriggerMode',{{2,'OFF',[1 3]}},'TriggerLineOut',{{1,'OFF',[1 16]}},'ADCSWStartEnable',{{0,'OFF',[0 1]}},'SampleTime',{{'-1','OFF',[-1 inf]}},'SampleTimeCheck',{{1,'OFF',[]}},'StatusPortEnable',{{0,'OFF',[0 1]}},'TLCFileName',{{'rti120xadc_c1_adc','OFF',[]}})  RTISFcnParameters=struct('ReadMode','int16','ChannelNo','int16','ConversionMode','int16','TriggerSource','int16','TriggerLineIn','int16','SampleMode','int16','BurstTriggerSource','int16','BurstTriggerLine','int16','ConvTriggerSource','int16','ConvTriggerLine','int16','ConvPeriod','double','BurstSize','int16','DataSetOffset','int16','DataSetLength','int16','EnableTriggerEvent','int16','TriggerMode','int16','TriggerLineOut','int16','ADCSWStartEnable','int16','SampleTime','double','StatusPortEnable','int16','TLCFileName','char')  RTIBlockParaDefault=struct('ReadMode',1,'ChannelNo',1,'ConversionMode',1,'TriggerSource',1,'TriggerLineIn',1,'SampleMode',1,'BurstTriggerSource',1,'BurstTriggerLine',1,'ConvTriggerSource',3,'ConvTriggerLine',1,'ConvPeriod',0.0001,'ConvPeriodCheck',0,'BurstSize',10,'BurstSizeCheck',0,'DataSetOffset',0,'DataSetOffsetCheck',0,'DataSetLength',1,'DataSetLengthCheck',0,'EnableTriggerEvent',0,'TriggerMode',2,'TriggerLineOut',1,'ADCSWStartEnable',0,'SampleTime',-1,'SampleTimeCheck',1,'StatusPortEnable',0,'TLCFileName','rti120xadc_c1_adc')
  ADC_CLASS1_BL7 : rti1202lib_adc_class1/ADC_CLASS1_BL1  Commented=on  DSProperties=struct('RTI',struct('Version',uint32(1),'BlockType',struct('isSLSource',uint8(1),'isSLSink',uint8(1),'isHWSource',uint8(0),'isHWSink',uint8(1),'isSetup',uint8(0),'isInline',uint8(1),'isNonInline',uint8(0),'isInterrupt',uint8(0),'isChannelwise',uint8(1)),'IOBoardType',{{'DS120X','STD','ADCC1'}},'UnitType','ADC','Identifier','ADC','DialogType','ML','BlockSet','NONE','SlaveProcessor','NONE'))  RTIBlockInterface=struct('InputPortsActive',0,'InputPortsWidth',int32(1),'InputPortsDataType',{{'SS_BOOLEAN'}},'InputPortsName',{{'Continue'}},'OutputPortsActive',[1 0],'OutputPortsWidth',int32([1 1]),'OutputPortsDataType',{{'SS_DOUBLE','SS_INT16'}},'OutputPortsName',{{'ADC','Status'}},'DialogFcn','rti120xstdadcc1adcgui','SampleTime',{{-1}},'InitLevel',3,'IconTransparency','on','BlockDisplay',{{['ADC CL1\nChannel: 21'],'center'}},'BlockName',struct('Token',{{'ADC_CLASS1_BL1'}}))  RTIBlockParameters=struct('ReadMode',{{1,'OFF',[1 2]}},'ChannelNo',{{21,'OFF',[]}},'ConversionMode',{{1,'OFF',[1 2]}},'TriggerSource',{{1,'OFF',[1 2]}},'TriggerLineIn',{{1,'OFF',[1 16]}},'SampleMode',{{1,'OFF',[1 2]}},'BurstTriggerSource',{{1,'OFF',[1 2]}},'BurstTriggerLine',{{1,'OFF',[1 16]}},'ConvTriggerSource',{{3,'OFF',[1 3]}},'ConvTriggerLine',{{1,'OFF',[1 16]}},'ConvPeriod',{{'100e-6','OFF',[1e-6 1.34]}},'ConvPeriodCheck',{{0,'OFF',[]}},'BurstSize',{{'10','OFF',[]}},'BurstSizeCheck',{{0,'OFF',[]}},'DataSetOffset',{{'0','OFF',[]}},'DataSetOffsetCheck',{{0,'OFF',[]}},'DataSetLength',{{'1','OFF',[]}},'DataSetLengthCheck',{{0,'OFF',[]}},'EnableTriggerEvent',{{0,'OFF',[0 1]}},'TriggerMode',{{2,'OFF',[1 3]}},'TriggerLineOut',{{1,'OFF',[1 16]}},'ADCSWStartEnable',{{0,'OFF',[0 1]}},'SampleTime',{{'-1','OFF',[-1 inf]}},'SampleTimeCheck',{{1,'OFF',[]}},'StatusPortEnable',{{0,'OFF',[0 1]}},'TLCFileName',{{'rti120xadc_c1_adc','OFF',[]}})  RTISFcnParameters=struct('ReadMode','int16','ChannelNo','int16','ConversionMode','int16','TriggerSource','int16','TriggerLineIn','int16','SampleMode','int16','BurstTriggerSource','int16','BurstTriggerLine','int16','ConvTriggerSource','int16','ConvTriggerLine','int16','ConvPeriod','double','BurstSize','int16','DataSetOffset','int16','DataSetLength','int16','EnableTriggerEvent','int16','TriggerMode','int16','TriggerLineOut','int16','ADCSWStartEnable','int16','SampleTime','double','StatusPortEnable','int16','TLCFileName','char')  RTIBlockParaDefault=struct('ReadMode',1,'ChannelNo',1,'ConversionMode',1,'TriggerSource',1,'TriggerLineIn',1,'SampleMode',1,'BurstTriggerSource',1,'BurstTriggerLine',1,'ConvTriggerSource',3,'ConvTriggerLine',1,'ConvPeriod',0.0001,'ConvPeriodCheck',0,'BurstSize',10,'BurstSizeCheck',0,'DataSetOffset',0,'DataSetOffsetCheck',0,'DataSetLength',1,'DataSetLengthCheck',0,'EnableTriggerEvent',0,'TriggerMode',2,'TriggerLineOut',1,'ADCSWStartEnable',0,'SampleTime',-1,'SampleTimeCheck',1,'StatusPortEnable',0,'TLCFileName','rti120xadc_c1_adc')
  ADC_CLASS1_BL8 : rti1202lib_adc_class1/ADC_CLASS1_BL1  Commented=on  DSProperties=struct('RTI',struct('Version',uint32(1),'BlockType',struct('isSLSource',uint8(1),'isSLSink',uint8(1),'isHWSource',uint8(0),'isHWSink',uint8(1),'isSetup',uint8(0),'isInline',uint8(1),'isNonInline',uint8(0),'isInterrupt',uint8(0),'isChannelwise',uint8(1)),'IOBoardType',{{'DS120X','STD','ADCC1'}},'UnitType','ADC','Identifier','ADC','DialogType','ML','BlockSet','NONE','SlaveProcessor','NONE'))  RTIBlockInterface=struct('InputPortsActive',0,'InputPortsWidth',int32(1),'InputPortsDataType',{{'SS_BOOLEAN'}},'InputPortsName',{{'Continue'}},'OutputPortsActive',[1 0],'OutputPortsWidth',int32([1 1]),'OutputPortsDataType',{{'SS_DOUBLE','SS_INT16'}},'OutputPortsName',{{'ADC','Status'}},'DialogFcn','rti120xstdadcc1adcgui','SampleTime',{{-1}},'InitLevel',3,'IconTransparency','on','BlockDisplay',{{['ADC CL1\nChannel: 20'],'center'}},'BlockName',struct('Token',{{'ADC_CLASS1_BL1'}}))  RTIBlockParameters=struct('ReadMode',{{1,'OFF',[1 2]}},'ChannelNo',{{20,'OFF',[]}},'ConversionMode',{{1,'OFF',[1 2]}},'TriggerSource',{{1,'OFF',[1 2]}},'TriggerLineIn',{{1,'OFF',[1 16]}},'SampleMode',{{1,'OFF',[1 2]}},'BurstTriggerSource',{{1,'OFF',[1 2]}},'BurstTriggerLine',{{1,'OFF',[1 16]}},'ConvTriggerSource',{{3,'OFF',[1 3]}},'ConvTriggerLine',{{1,'OFF',[1 16]}},'ConvPeriod',{{'100e-6','OFF',[1e-6 1.34]}},'ConvPeriodCheck',{{0,'OFF',[]}},'BurstSize',{{'10','OFF',[]}},'BurstSizeCheck',{{0,'OFF',[]}},'DataSetOffset',{{'0','OFF',[]}},'DataSetOffsetCheck',{{0,'OFF',[]}},'DataSetLength',{{'1','OFF',[]}},'DataSetLengthCheck',{{0,'OFF',[]}},'EnableTriggerEvent',{{0,'OFF',[0 1]}},'TriggerMode',{{2,'OFF',[1 3]}},'TriggerLineOut',{{1,'OFF',[1 16]}},'ADCSWStartEnable',{{0,'OFF',[0 1]}},'SampleTime',{{'-1','OFF',[-1 inf]}},'SampleTimeCheck',{{1,'OFF',[]}},'StatusPortEnable',{{0,'OFF',[0 1]}},'TLCFileName',{{'rti120xadc_c1_adc','OFF',[]}})  RTISFcnParameters=struct('ReadMode','int16','ChannelNo','int16','ConversionMode','int16','TriggerSource','int16','TriggerLineIn','int16','SampleMode','int16','BurstTriggerSource','int16','BurstTriggerLine','int16','ConvTriggerSource','int16','ConvTriggerLine','int16','ConvPeriod','double','BurstSize','int16','DataSetOffset','int16','DataSetLength','int16','EnableTriggerEvent','int16','TriggerMode','int16','TriggerLineOut','int16','ADCSWStartEnable','int16','SampleTime','double','StatusPortEnable','int16','TLCFileName','char')  RTIBlockParaDefault=struct('ReadMode',1,'ChannelNo',1,'ConversionMode',1,'TriggerSource',1,'TriggerLineIn',1,'SampleMode',1,'BurstTriggerSource',1,'BurstTriggerLine',1,'ConvTriggerSource',3,'ConvTriggerLine',1,'ConvPeriod',0.0001,'ConvPeriodCheck',0,'BurstSize',10,'BurstSizeCheck',0,'DataSetOffset',0,'DataSetOffsetCheck',0,'DataSetLength',1,'DataSetLengthCheck',0,'EnableTriggerEvent',0,'TriggerMode',2,'TriggerLineOut',1,'ADCSWStartEnable',0,'SampleTime',-1,'SampleTimeCheck',1,'StatusPortEnable',0,'TLCFileName','rti120xadc_c1_adc')
  AO_f_ow : Constant  Commented=on  Value=0
  AO_r_ow : Constant  Commented=on  Value=0
  Add{,7,11..12} (4 alike) : Sum
  Add10 : Sum  Commented=on
  Add15 : Sum  Commented=on  Inputs=+++
  Add{2..6} (5 alike) : Sum  Inputs=+-
  Add21 : Sum  Commented=on  Inputs=+++
  Ao_release_current : From  Commented=on  GotoTag=Ao_release_input_Current  TagVisibility=global
  Ao_tank_fill_current : From  Commented=on  GotoTag=Ao_Fill_current  TagVisibility=global
  Bar2Pa{,1..6} (7 alike) : Gain  Gain=100000
  Bias1 : Bias  Commented=on  Bias=-0.0011  SaturateOnIntegerOverflow=off
  Bias10 : Bias  Bias=-23.3727-203.3199  SaturateOnIntegerOverflow=off
  Bias11 : Bias  Bias=138.9018-399.1358  SaturateOnIntegerOverflow=off
  Bias3 : Bias  Commented=on  Bias=-0.1054  SaturateOnIntegerOverflow=off
  Bias4 : Bias  Commented=on  Bias=-0.1138  SaturateOnIntegerOverflow=off
  Bias8 : Bias  Bias=-281.4181--6.2469  SaturateOnIntegerOverflow=off
  Bias9 : Bias  Bias=-275.4219-25.4399  SaturateOnIntegerOverflow=off
  CVS_on_off : Constant
  Clock3 : Clock  Commented=on
  Clock4 : Clock  Commented=on
  Compare To Zero : simulink/Logic and Bit Operations/Compare To Zero  Commented=on  relop=<=  OutDataTypeStr=boolean
  Compressor to P1 Fill : MATLAB Function  TreatAsAtomicUnit=on
  Constant : Constant  Commented=on  Value=0
  Constant{1,3..6,15} (6 alike) : Constant  Value=0
  Constant11 : Constant  Commented=on
  Constant12 : Constant  Commented=on
  Constant2 : Constant  Commented=on  Value=0.2
  Constant20 : Constant  Commented=on  Value=120
  Constant21 : Constant  Commented=on  Value=8
  DAC_CLASS1_BL1 : rti1202lib_dac_class1/DAC_CLASS1_BL1  Commented=on  DSProperties=struct('RTI',struct('Version',uint32(2),'BlockType',struct('isSLSource',uint8(0),'isSLSink',uint8(1),'isHWSource',uint8(0),'isHWSink',uint8(1),'isSetup',uint8(0),'isInline',uint8(1),'isNonInline',uint8(0),'isInterrupt',uint8(0),'isChannelwise',uint8(1)),'IOBoardType',{{'DS120X','STD','DACC1'}},'UnitType','DAC','Identifier','DAC','DialogType','ML','BlockSet','NONE','SlaveProcessor','NONE'))  RTIBlockInterface=struct('InputPortsActive',1,'InputPortsWidth',int32(1),'InputPortsDataType',{{'SS_DOUBLE'}},'InputPortsName',{{['DAC 2']}},'DialogFcn','rti120xstddacc1dacgui','InitLevel',3,'IconTransparency','on','BlockDisplay',{{['DAC CL1\nChannel: 2'],'center'}},'BlockName',struct('Token',{{'DAC_CLASS1_BL1'}}))  RTIBlockParameters=struct('ChannelNo',{{2,'OFF',[]}},'ChannelNumOf',{{1,'OFF',[]}},'InitialValue1',{{'0','OFF',[-10 10]}},'InitialValue2',{{'0','OFF',[-10 10]}},'InitialValue3',{{'0','OFF',[-10 10]}},'InitialValue4',{{'0','OFF',[-10 10]}},'InitialValue5',{{'0','OFF',[-10 10]}},'InitialValue6',{{'0','OFF',[-10 10]}},'InitialValue7',{{'0','OFF',[-10 10]}},'InitialValue8',{{'0','OFF',[-10 10]}},'InitialValue9',{{'0','OFF',[-10 10]}},'InitialValue10',{{'0','OFF',[-10 10]}},'InitialValue11',{{'0','OFF',[-10 10]}},'InitialValue12',{{'0','OFF',[-10 10]}},'InitialValue13',{{'0','OFF',[-10 10]}},'InitialValue14',{{'0','OFF',[-10 10]}},'InitialValue15',{{'0','OFF',[-10 10]}},'InitialValue16',{{'0','OFF',[-10 10]}},'OutputMode',{{ones(1,16),'OFF',[1 2]}},'TermValue1',{{'0','OFF',[-10 10]}},'TermValue2',{{'0','OFF',[-10 10]}},'TermValue3',{{'0','OFF',[-10 10]}},'TermValue4',{{'0','OFF',[-10 10]}},'TermValue5',{{'0','OFF',[-10 10]}},'TermValue6',{{'0','OFF',[-10 10]}},'TermValue7',{{'0','OFF',[-10 10]}},'TermValue8',{{'0','OFF',[-10 10]}},'TermValue9',{{'0','OFF',[-10 10]}},'TermValue10',{{'0','OFF',[-10 10]}},'TermValue11',{{'0','OFF',[-10 10]}},'TermValue12',{{'0','OFF',[-10 10]}},'TermValue13',{{'0','OFF',[-10 10]}},'TermValue14',{{'0','OFF',[-10 10]}},'TermValue15',{{'0','OFF',[-10 10]}},'TermValue16',{{'0','OFF',[-10 10]}},'EnableTermMode',{{0,'OFF',[0 1]}},'TLCFileName',{{'rti120xdac_c1_dac','OFF',[]}},'InitialValueBuildCheck1',{{0,'OFF',[]}},'InitialValueBuildCheck2',{{1,'OFF',[]}},'InitialValueBuildCheck3',{{0,'OFF',[]}},'InitialValueBuildCheck4',{{0,'OFF',[]}},'InitialValueBuildCheck5',{{0,'OFF',[]}},'InitialValueBuildCheck6',{{0,'OFF',[]}},'InitialValueBuildCheck7',{{0,'OFF',[]}},'InitialValueBuildCheck8',{{0,'OFF',[]}},'InitialValueBuildCheck9',{{0,'OFF',[]}},'InitialValueBuildCheck10',{{0,'OFF',[]}},'InitialValueBuildCheck11',{{0,'OFF',[]}},'InitialValueBuildCheck12',{{0,'OFF',[]}},'InitialValueBuildCheck13',{{0,'OFF',[]}},'InitialValueBuildCheck14',{{0,'OFF',[]}},'InitialValueBuildCheck15',{{0,'OFF',[]}},'InitialValueBuildCheck16',{{0,'OFF',[]}},'TermValueBuildCheck1',{{0,'OFF',[]}},'TermValueBuildCheck2',{{0,'OFF',[]}},'TermValueBuildCheck3',{{0,'OFF',[]}},'TermValueBuildCheck4',{{0,'OFF',[]}},'TermValueBuildCheck5',{{0,'OFF',[]}},'TermValueBuildCheck6',{{0,'OFF',[]}},'TermValueBuildCheck7',{{0,'OFF',[]}},'TermValueBuildCheck8',{{0,'OFF',[]}},'TermValueBuildCheck9',{{0,'OFF',[]}},'TermValueBuildCheck10',{{0,'OFF',[]}},'TermValueBuildCheck11',{{0,'OFF',[]}},'TermValueBuildCheck12',{{0,'OFF',[]}},'TermValueBuildCheck13',{{0,'OFF',[]}},'TermValueBuildCheck14',{{0,'OFF',[]}},'TermValueBuildCheck15',{{0,'OFF',[]}},'TermValueBuildCheck16',{{0,'OFF',[]}})  RTISFcnParameters=struct('ChannelNo','int16','ChannelNumOf','int16','InitialValue1','double','InitialValue2','double','InitialValue3','double','InitialValue4','double','InitialValue5','double','InitialValue6','double','InitialValue7','double','InitialValue8','double','InitialValue9','double','InitialValue10','double','InitialValue11','double','InitialValue12','double','InitialValue13','double','InitialValue14','double','InitialValue15','double','InitialValue16','double','OutputMode','int16','TermValue1','double','TermValue2','double','TermValue3','double','TermValue4','double','TermValue5','double','TermValue6','double','TermValue7','double','TermValue8','double','TermValue9','double','TermValue10','double','TermValue11','double','TermValue12','double','TermValue13','double','TermValue14','double','TermValue15','double','TermValue16','double','EnableTermMode','int16','TLCFileName','char')  RTIBlockParaDefault=struct('ChannelNo',1,'ChannelNumOf',1,'InitialValue1',0,'InitialValue2',0,'InitialValue3',0,'InitialValue4',0,'InitialValue5',0,'InitialValue6',0,'InitialValue7',0,'InitialValue8',0,'InitialValue9',0,'InitialValue10',0,'InitialValue11',0,'InitialValue12',0,'InitialValue13',0,'InitialValue14',0,'InitialValue15',0,'InitialValue16',0,'OutputMode',ones(1,16),'TermValue1',0,'TermValue2',0,'TermValue3',0,'TermValue4',0,'TermValue5',0,'TermValue6',0,'TermValue7',0,'TermValue8',0,'TermValue9',0,'TermValue10',0,'TermValue11',0,'TermValue12',0,'TermValue13',0,'TermValue14',0,'TermValue15',0,'TermValue16',0,'EnableTermMode',0,'TLCFileName','rti120xdac_c1_dac','InitialValueBuildCheck1',0,'InitialValueBuildCheck2',0,'InitialValueBuildCheck3',0,'InitialValueBuildCheck4',0,'InitialValueBuildCheck5',0,'InitialValueBuildCheck6',0,'InitialValueBuildCheck7',0,'InitialValueBuildCheck8',0,'InitialValueBuildCheck9',0,'InitialValueBuildCheck10',0,'InitialValueBuildCheck11',0,'InitialValueBuildCheck12',0,'InitialValueBuildCheck13',0,'InitialValueBuildCheck14',0,'InitialValueBuildCheck15',0,'InitialValueBuildCheck16',0,'TermValueBuildCheck1',0,'TermValueBuildCheck2',0,'TermValueBuildCheck3',0,'TermValueBuildCheck4',0,'TermValueBuildCheck5',0,'TermValueBuildCheck6',0,'TermValueBuildCheck7',0,'TermValueBuildCheck8',0,'TermValueBuildCheck9',0,'TermValueBuildCheck10',0,'TermValueBuildCheck11',0,'TermValueBuildCheck12',0,'TermValueBuildCheck13',0,'TermValueBuildCheck14',0,'TermValueBuildCheck15',0,'TermValueBuildCheck16',0)
  DIO_CLASS1_BIT_OUT_BL1 : rti1202lib_dio_class1/DIO_CLASS1_BIT_OUT_BL1  Commented=on  DSProperties=struct('RTI',struct('Version',uint32(1),'BlockType',struct('isSLSource',uint8(0),'isSLSink',uint8(1),'isHWSource',uint8(0),'isHWSink',uint8(1),'isSetup',uint8(0),'isInline',uint8(1),'isNonInline',uint8(0),'isInterrupt',uint8(0),'isChannelwise',uint8(1)),'IOBoardType',{{'DS120X','STD','DIOC1'}},'UnitType','BIT','Identifier','BITOUT','DialogType','ML','BlockSet','NONE','SlaveProcessor','NONE'))  RTIBlockInterface=struct('InputPortsWidth',int32(1),'InputPortsActive',1,'InputPortsDataType',{{'SS_BOOLEAN'}},'InputPortsName',{{'In'}},'BlockDisplay',{{['DIO CL1 BIT OUT\nPort: 2\nChannel: 16\nNumber of channels: 1'],'center\'}},'IconTransparency','on','InitLevel',3,'DialogFcn','rti120xstddioc1bitoutgui','BlockName',struct('Token',{{'DIO_CLASS1_BIT_OUT_BL1'}}))  RTIBlockParameters=struct('PortNo',{{2,'OFF',[]}},'ChannelNo',{{16,'OFF',[]}},'ChannelNumOf',{{1,'OFF',[]}},'HighLevel',{{3,'OFF',[1 3]}},'OutputStateInit',{{zeros(1,16),'OFF',[0 1]}},'OutputStateTerm',{{zeros(1,16),'OFF',[0 1]}},'TerminationMode',{{0,'OFF',[0 1]}},'OutputStateTermValidate',{{0,'OFF',[0 1]}},'OutputStateInitSetAll',{{0,'OFF',[0 1]}},'OutputStateTermSetAll',{{0,'OFF',[0 1]}},'EnableEvent',{{0,'OFF',[0 1]}},'EventMode',{{1,'OFF',[1 3]}},'EventOnFalling',{{1,'OFF',[0 1]}},'EventOnRising',{{0,'OFF',[0 1]}},'EventDelay',{{'0','OFF',[0 1.34]}},'EventRate',{{'1','OFF',[1 256]}},'EventBuildCheck',{{false,'OFF',[]}},'TriggerLine',{{1,'OFF',[1 16]}},'EventChannelNoIdx',{{1,'OFF',[1 16]}},'TLCFileName',{{'rti120xdio_c1_bit_out','OFF',[]}})  RTISFcnParameters=struct('PortNo','int16','ChannelNo','int16','ChannelNumOf','int16','HighLevel','int16','OutputStateInit','int16','OutputStateTerm','int16','TerminationMode','int16','OutputStateTermValidate','int16','EnableEvent','int16','EventMode','int16','EventOnFalling','int16','EventOnRising','int16','EventDelay','double','EventRate','int16','TriggerLine','int16','EventChannelNoIdx','int16','TLCFileName','char')  RTIBlockParaDefault=struct('PortNo',1,'ChannelNo',1,'ChannelNumOf',1,'HighLevel',1,'OutputStateInit',zeros(1,16),'OutputStateTerm',zeros(1,16),'TerminationMode',0,'OutputStateTermValidate',0,'OutputStateInitSetAll',0,'OutputStateTermSetAll',0,'EnableEvent',0,'EventMode',1,'EventOnFalling',1,'EventOnRising',0,'EventDelay',0,'EventRate',1,'EventBuildCheck',0,'TriggerLine',1,'EventChannelNoIdx',1,'TLCFileName','rti120xdio_c1_bit_out')
  DIO_CLASS1_PWM_BL1 : rti1202lib_dio_class1/DIO_CLASS1_PWM_BL1  Commented=on  DSProperties=struct('RTI',struct('Version',uint32(1),'BlockType',struct('isSLSource',uint8(0),'isSLSink',uint8(1),'isHWSource',uint8(0),'isHWSink',uint8(1),'isSetup',uint8(0),'isInline',uint8(1),'isNonInline',uint8(0),'isInterrupt',uint8(0),'isChannelwise',uint8(1)),'IOBoardType',{{'DS120X','STD','DIOC1'}},'UnitType','PWM','Identifier','PWM','DialogType','ML','BlockSet','NONE','SlaveProcessor','NONE'))  RTIBlockInterface=struct('InputPortsWidth',int32([1 1]),'InputPortsActive',[1 1],'InputPortsName',{{'Period',['Duty Cycle']}},'BlockDisplay',{{['DIO CL1 PWM\nPort: 1\nChannel: 4'],'center'}},'IconTransparency','on','InitLevel',3,'DialogFcn','rti120xstddioc1pwmgui','BlockName',struct('Token',{{'DIO_CLASS1_PWM_BL1'}}))  RTIBlockParameters=struct('PortNo',{{1,'OFF',[]}},'ChannelNo',{{4,'OFF',[]}},'HighLevel',{{3,'OFF',[1 3]}},'UpdateMode',{{1,'OFF',[1 2]}},'InvertingMode',{{1,'OFF',[1 2]}},'DutyCycleInit',{{'0.5','OFF',[0 1]}},'DutyCycleTerm',{{'0.5','OFF',[0 1]}},'PeriodInit',{{'5e-05','OFF',[1e-7 1.34]}},'PeriodTerm',{{'5e-05','OFF',[1e-7 1.34]}},'TerminationMode',{{0,'OFF',[0 1]}},'OutputTermValidate',{{0,'OFF',[0 1]}},'OutputTermBuildCheck',{{false,'OFF',[]}},'EnableEvent',{{0,'OFF',[0 1]}},'EventMode',{{1,'OFF',[1 3]}},'EventOnFalling',{{1,'OFF',[0 1]}},'EventOnRising',{{0,'OFF',[0 1]}},'EventDelay',{{'0','OFF',[0 1.34]}},'EventRate',{{'1','OFF',[1 256]}},'EventBuildCheck',{{false,'OFF',[]}},'TriggerLine',{{1,'OFF',[1 16]}},'TLCFileName',{{'rti120xdio_c1_pwm','OFF',[]}})  RTISFcnParameters=struct('PortNo','int16','ChannelNo','int16','HighLevel','int16','UpdateMode','int16','InvertingMode','int16','DutyCycleInit','double','DutyCycleTerm','double','PeriodInit','double','PeriodTerm','double','TerminationMode','int16','OutputTermValidate','int16','EnableEvent','int16','EventMode','int16','EventOnFalling','int16','EventOnRising','int16','EventDelay','double','EventRate','int16','TriggerLine','int16','TLCFileName','char')  RTIBlockParaDefault=struct('PortNo',1,'ChannelNo',1,'HighLevel',1,'UpdateMode',1,'InvertingMode',1,'DutyCycleInit',2^-1,'DutyCycleTerm',2^-1,'PeriodInit',5e-5,'PeriodTerm',5e-5,'TerminationMode',0,'OutputTermValidate',0,'OutputTermBuildCheck',0,'EnableEvent',0,'EventMode',1,'EventOnFalling',1,'EventOnRising',0,'EventDelay',0,'EventRate',1,'EventBuildCheck',0,'TriggerLine',1,'TLCFileName','rti120xdio_c1_pwm')
  DIO_CLASS1_PWM_BL2 : rti1202lib_dio_class1/DIO_CLASS1_PWM_BL1  Commented=on  DSProperties=struct('RTI',struct('Version',uint32(1),'BlockType',struct('isSLSource',uint8(0),'isSLSink',uint8(1),'isHWSource',uint8(0),'isHWSink',uint8(1),'isSetup',uint8(0),'isInline',uint8(1),'isNonInline',uint8(0),'isInterrupt',uint8(0),'isChannelwise',uint8(1)),'IOBoardType',{{'DS120X','STD','DIOC1'}},'UnitType','PWM','Identifier','PWM','DialogType','ML','BlockSet','NONE','SlaveProcessor','NONE'))  RTIBlockInterface=struct('InputPortsWidth',int32([1 1]),'InputPortsActive',[1 1],'InputPortsName',{{'Period',['Duty Cycle']}},'BlockDisplay',{{['DIO CL1 PWM\nPort: 1\nChannel: 6'],'center'}},'IconTransparency','on','InitLevel',3,'DialogFcn','rti120xstddioc1pwmgui','BlockName',struct('Token',{{'DIO_CLASS1_PWM_BL1'}}))  RTIBlockParameters=struct('PortNo',{{1,'OFF',[]}},'ChannelNo',{{6,'OFF',[]}},'HighLevel',{{3,'OFF',[1 3]}},'UpdateMode',{{1,'OFF',[1 2]}},'InvertingMode',{{1,'OFF',[1 2]}},'DutyCycleInit',{{'0.5','OFF',[0 1]}},'DutyCycleTerm',{{'0.5','OFF',[0 1]}},'PeriodInit',{{'5e-05','OFF',[1e-7 1.34]}},'PeriodTerm',{{'5e-05','OFF',[1e-7 1.34]}},'TerminationMode',{{0,'OFF',[0 1]}},'OutputTermValidate',{{0,'OFF',[0 1]}},'OutputTermBuildCheck',{{false,'OFF',[]}},'EnableEvent',{{0,'OFF',[0 1]}},'EventMode',{{1,'OFF',[1 3]}},'EventOnFalling',{{1,'OFF',[0 1]}},'EventOnRising',{{0,'OFF',[0 1]}},'EventDelay',{{'0','OFF',[0 1.34]}},'EventRate',{{'1','OFF',[1 256]}},'EventBuildCheck',{{false,'OFF',[]}},'TriggerLine',{{1,'OFF',[1 16]}},'TLCFileName',{{'rti120xdio_c1_pwm','OFF',[]}})  RTISFcnParameters=struct('PortNo','int16','ChannelNo','int16','HighLevel','int16','UpdateMode','int16','InvertingMode','int16','DutyCycleInit','double','DutyCycleTerm','double','PeriodInit','double','PeriodTerm','double','TerminationMode','int16','OutputTermValidate','int16','EnableEvent','int16','EventMode','int16','EventOnFalling','int16','EventOnRising','int16','EventDelay','double','EventRate','int16','TriggerLine','int16','TLCFileName','char')  RTIBlockParaDefault=struct('PortNo',1,'ChannelNo',1,'HighLevel',1,'UpdateMode',1,'InvertingMode',1,'DutyCycleInit',2^-1,'DutyCycleTerm',2^-1,'PeriodInit',5e-5,'PeriodTerm',5e-5,'TerminationMode',0,'OutputTermValidate',0,'OutputTermBuildCheck',0,'EnableEvent',0,'EventMode',1,'EventOnFalling',1,'EventOnRising',0,'EventDelay',0,'EventRate',1,'EventBuildCheck',0,'TriggerLine',1,'TLCFileName','rti120xdio_c1_pwm')
  DIO_CLASS1_PWM_BL3 : rti1202lib_dio_class1/DIO_CLASS1_PWM_BL1  Commented=on  DSProperties=struct('RTI',struct('Version',uint32(1),'BlockType',struct('isSLSource',uint8(0),'isSLSink',uint8(1),'isHWSource',uint8(0),'isHWSink',uint8(1),'isSetup',uint8(0),'isInline',uint8(1),'isNonInline',uint8(0),'isInterrupt',uint8(0),'isChannelwise',uint8(1)),'IOBoardType',{{'DS120X','STD','DIOC1'}},'UnitType','PWM','Identifier','PWM','DialogType','ML','BlockSet','NONE','SlaveProcessor','NONE'))  RTIBlockInterface=struct('InputPortsWidth',int32([1 1]),'InputPortsActive',[1 1],'InputPortsName',{{'Period',['Duty Cycle']}},'BlockDisplay',{{['DIO CL1 PWM\nPort: 1\nChannel: 1'],'center'}},'IconTransparency','on','InitLevel',3,'DialogFcn','rti120xstddioc1pwmgui','BlockName',struct('Token',{{'DIO_CLASS1_PWM_BL1'}}))  RTIBlockParameters=struct('PortNo',{{1,'OFF',[]}},'ChannelNo',{{1,'OFF',[]}},'HighLevel',{{3,'OFF',[1 3]}},'UpdateMode',{{1,'OFF',[1 2]}},'InvertingMode',{{1,'OFF',[1 2]}},'DutyCycleInit',{{'0.5','OFF',[0 1]}},'DutyCycleTerm',{{'0.5','OFF',[0 1]}},'PeriodInit',{{'5e-05','OFF',[1e-7 1.34]}},'PeriodTerm',{{'5e-05','OFF',[1e-7 1.34]}},'TerminationMode',{{0,'OFF',[0 1]}},'OutputTermValidate',{{0,'OFF',[0 1]}},'OutputTermBuildCheck',{{false,'OFF',[]}},'EnableEvent',{{0,'OFF',[0 1]}},'EventMode',{{1,'OFF',[1 3]}},'EventOnFalling',{{1,'OFF',[0 1]}},'EventOnRising',{{0,'OFF',[0 1]}},'EventDelay',{{'0','OFF',[0 1.34]}},'EventRate',{{'1','OFF',[1 256]}},'EventBuildCheck',{{false,'OFF',[]}},'TriggerLine',{{1,'OFF',[1 16]}},'TLCFileName',{{'rti120xdio_c1_pwm','OFF',[]}})  RTISFcnParameters=struct('PortNo','int16','ChannelNo','int16','HighLevel','int16','UpdateMode','int16','InvertingMode','int16','DutyCycleInit','double','DutyCycleTerm','double','PeriodInit','double','PeriodTerm','double','TerminationMode','int16','OutputTermValidate','int16','EnableEvent','int16','EventMode','int16','EventOnFalling','int16','EventOnRising','int16','EventDelay','double','EventRate','int16','TriggerLine','int16','TLCFileName','char')  RTIBlockParaDefault=struct('PortNo',1,'ChannelNo',1,'HighLevel',1,'UpdateMode',1,'InvertingMode',1,'DutyCycleInit',2^-1,'DutyCycleTerm',2^-1,'PeriodInit',5e-5,'PeriodTerm',5e-5,'TerminationMode',0,'OutputTermValidate',0,'OutputTermBuildCheck',0,'EnableEvent',0,'EventMode',1,'EventOnFalling',1,'EventOnRising',0,'EventDelay',0,'EventRate',1,'EventBuildCheck',0,'TriggerLine',1,'TLCFileName','rti120xdio_c1_pwm')
  DIO_CLASS1_PWM_BL4 : rti1202lib_dio_class1/DIO_CLASS1_PWM_BL1  Commented=on  DSProperties=struct('RTI',struct('Version',uint32(1),'BlockType',struct('isSLSource',uint8(0),'isSLSink',uint8(1),'isHWSource',uint8(0),'isHWSink',uint8(1),'isSetup',uint8(0),'isInline',uint8(1),'isNonInline',uint8(0),'isInterrupt',uint8(0),'isChannelwise',uint8(1)),'IOBoardType',{{'DS120X','STD','DIOC1'}},'UnitType','PWM','Identifier','PWM','DialogType','ML','BlockSet','NONE','SlaveProcessor','NONE'))  RTIBlockInterface=struct('InputPortsWidth',int32([1 1]),'InputPortsActive',[1 1],'InputPortsName',{{'Period',['Duty Cycle']}},'BlockDisplay',{{['DIO CL1 PWM\nPort: 1\nChannel: 8'],'center'}},'IconTransparency','on','InitLevel',3,'DialogFcn','rti120xstddioc1pwmgui','BlockName',struct('Token',{{'DIO_CLASS1_PWM_BL1'}}))  RTIBlockParameters=struct('PortNo',{{1,'OFF',[]}},'ChannelNo',{{8,'OFF',[]}},'HighLevel',{{3,'OFF',[1 3]}},'UpdateMode',{{1,'OFF',[1 2]}},'InvertingMode',{{1,'OFF',[1 2]}},'DutyCycleInit',{{'0.5','OFF',[0 1]}},'DutyCycleTerm',{{'0.5','OFF',[0 1]}},'PeriodInit',{{'5e-05','OFF',[1e-7 1.34]}},'PeriodTerm',{{'5e-05','OFF',[1e-7 1.34]}},'TerminationMode',{{0,'OFF',[0 1]}},'OutputTermValidate',{{0,'OFF',[0 1]}},'OutputTermBuildCheck',{{false,'OFF',[]}},'EnableEvent',{{0,'OFF',[0 1]}},'EventMode',{{1,'OFF',[1 3]}},'EventOnFalling',{{1,'OFF',[0 1]}},'EventOnRising',{{0,'OFF',[0 1]}},'EventDelay',{{'0','OFF',[0 1.34]}},'EventRate',{{'1','OFF',[1 256]}},'EventBuildCheck',{{false,'OFF',[]}},'TriggerLine',{{1,'OFF',[1 16]}},'TLCFileName',{{'rti120xdio_c1_pwm','OFF',[]}})  RTISFcnParameters=struct('PortNo','int16','ChannelNo','int16','HighLevel','int16','UpdateMode','int16','InvertingMode','int16','DutyCycleInit','double','DutyCycleTerm','double','PeriodInit','double','PeriodTerm','double','TerminationMode','int16','OutputTermValidate','int16','EnableEvent','int16','EventMode','int16','EventOnFalling','int16','EventOnRising','int16','EventDelay','double','EventRate','int16','TriggerLine','int16','TLCFileName','char')  RTIBlockParaDefault=struct('PortNo',1,'ChannelNo',1,'HighLevel',1,'UpdateMode',1,'InvertingMode',1,'DutyCycleInit',2^-1,'DutyCycleTerm',2^-1,'PeriodInit',5e-5,'PeriodTerm',5e-5,'TerminationMode',0,'OutputTermValidate',0,'OutputTermBuildCheck',0,'EnableEvent',0,'EventMode',1,'EventOnFalling',1,'EventOnRising',0,'EventDelay',0,'EventRate',1,'EventBuildCheck',0,'TriggerLine',1,'TLCFileName','rti120xdio_c1_pwm')
  DIO_CLASS1_PWM_BL6 : rti1202lib_dio_class1/DIO_CLASS1_PWM_BL1  Commented=on  DSProperties=struct('RTI',struct('Version',uint32(1),'BlockType',struct('isSLSource',uint8(0),'isSLSink',uint8(1),'isHWSource',uint8(0),'isHWSink',uint8(1),'isSetup',uint8(0),'isInline',uint8(1),'isNonInline',uint8(0),'isInterrupt',uint8(0),'isChannelwise',uint8(1)),'IOBoardType',{{'DS120X','STD','DIOC1'}},'UnitType','PWM','Identifier','PWM','DialogType','ML','BlockSet','NONE','SlaveProcessor','NONE'))  RTIBlockInterface=struct('InputPortsWidth',int32([1 1]),'InputPortsActive',[1 1],'InputPortsName',{{'Period',['Duty Cycle']}},'BlockDisplay',{{['DIO CL1 PWM\nPort: 1\nChannel: 5'],'center'}},'IconTransparency','on','InitLevel',3,'DialogFcn','rti120xstddioc1pwmgui','BlockName',struct('Token',{{'DIO_CLASS1_PWM_BL1'}}))  RTIBlockParameters=struct('PortNo',{{1,'OFF',[]}},'ChannelNo',{{5,'OFF',[]}},'HighLevel',{{3,'OFF',[1 3]}},'UpdateMode',{{1,'OFF',[1 2]}},'InvertingMode',{{1,'OFF',[1 2]}},'DutyCycleInit',{{'0.5','OFF',[0 1]}},'DutyCycleTerm',{{'0.5','OFF',[0 1]}},'PeriodInit',{{'5e-05','OFF',[1e-7 1.34]}},'PeriodTerm',{{'5e-05','OFF',[1e-7 1.34]}},'TerminationMode',{{0,'OFF',[0 1]}},'OutputTermValidate',{{0,'OFF',[0 1]}},'OutputTermBuildCheck',{{false,'OFF',[]}},'EnableEvent',{{0,'OFF',[0 1]}},'EventMode',{{1,'OFF',[1 3]}},'EventOnFalling',{{1,'OFF',[0 1]}},'EventOnRising',{{0,'OFF',[0 1]}},'EventDelay',{{'0','OFF',[0 1.34]}},'EventRate',{{'1','OFF',[1 256]}},'EventBuildCheck',{{false,'OFF',[]}},'TriggerLine',{{1,'OFF',[1 16]}},'TLCFileName',{{'rti120xdio_c1_pwm','OFF',[]}})  RTISFcnParameters=struct('PortNo','int16','ChannelNo','int16','HighLevel','int16','UpdateMode','int16','InvertingMode','int16','DutyCycleInit','double','DutyCycleTerm','double','PeriodInit','double','PeriodTerm','double','TerminationMode','int16','OutputTermValidate','int16','EnableEvent','int16','EventMode','int16','EventOnFalling','int16','EventOnRising','int16','EventDelay','double','EventRate','int16','TriggerLine','int16','TLCFileName','char')  RTIBlockParaDefault=struct('PortNo',1,'ChannelNo',1,'HighLevel',1,'UpdateMode',1,'InvertingMode',1,'DutyCycleInit',2^-1,'DutyCycleTerm',2^-1,'PeriodInit',5e-5,'PeriodTerm',5e-5,'TerminationMode',0,'OutputTermValidate',0,'OutputTermBuildCheck',0,'EnableEvent',0,'EventMode',1,'EventOnFalling',1,'EventOnRising',0,'EventDelay',0,'EventRate',1,'EventBuildCheck',0,'TriggerLine',1,'TLCFileName','rti120xdio_c1_pwm')
  DIO_CLASS1_PWM_BL7 : rti1202lib_dio_class1/DIO_CLASS1_PWM_BL1  Commented=on  DSProperties=struct('RTI',struct('Version',uint32(1),'BlockType',struct('isSLSource',uint8(0),'isSLSink',uint8(1),'isHWSource',uint8(0),'isHWSink',uint8(1),'isSetup',uint8(0),'isInline',uint8(1),'isNonInline',uint8(0),'isInterrupt',uint8(0),'isChannelwise',uint8(1)),'IOBoardType',{{'DS120X','STD','DIOC1'}},'UnitType','PWM','Identifier','PWM','DialogType','ML','BlockSet','NONE','SlaveProcessor','NONE'))  RTIBlockInterface=struct('InputPortsWidth',int32([1 1]),'InputPortsActive',[1 1],'InputPortsName',{{'Period',['Duty Cycle']}},'BlockDisplay',{{['DIO CL1 PWM\nPort: 1\nChannel: 13'],'center'}},'IconTransparency','on','InitLevel',3,'DialogFcn','rti120xstddioc1pwmgui','BlockName',struct('Token',{{'DIO_CLASS1_PWM_BL1'}}))  RTIBlockParameters=struct('PortNo',{{1,'OFF',[]}},'ChannelNo',{{13,'OFF',[]}},'HighLevel',{{3,'OFF',[1 3]}},'UpdateMode',{{1,'OFF',[1 2]}},'InvertingMode',{{1,'OFF',[1 2]}},'DutyCycleInit',{{'0.5','OFF',[0 1]}},'DutyCycleTerm',{{'0.5','OFF',[0 1]}},'PeriodInit',{{'5e-05','OFF',[1e-7 1.34]}},'PeriodTerm',{{'5e-05','OFF',[1e-7 1.34]}},'TerminationMode',{{0,'OFF',[0 1]}},'OutputTermValidate',{{0,'OFF',[0 1]}},'OutputTermBuildCheck',{{false,'OFF',[]}},'EnableEvent',{{0,'OFF',[0 1]}},'EventMode',{{1,'OFF',[1 3]}},'EventOnFalling',{{1,'OFF',[0 1]}},'EventOnRising',{{0,'OFF',[0 1]}},'EventDelay',{{'0','OFF',[0 1.34]}},'EventRate',{{'1','OFF',[1 256]}},'EventBuildCheck',{{false,'OFF',[]}},'TriggerLine',{{1,'OFF',[1 16]}},'TLCFileName',{{'rti120xdio_c1_pwm','OFF',[]}})  RTISFcnParameters=struct('PortNo','int16','ChannelNo','int16','HighLevel','int16','UpdateMode','int16','InvertingMode','int16','DutyCycleInit','double','DutyCycleTerm','double','PeriodInit','double','PeriodTerm','double','TerminationMode','int16','OutputTermValidate','int16','EnableEvent','int16','EventMode','int16','EventOnFalling','int16','EventOnRising','int16','EventDelay','double','EventRate','int16','TriggerLine','int16','TLCFileName','char')  RTIBlockParaDefault=struct('PortNo',1,'ChannelNo',1,'HighLevel',1,'UpdateMode',1,'InvertingMode',1,'DutyCycleInit',2^-1,'DutyCycleTerm',2^-1,'PeriodInit',5e-5,'PeriodTerm',5e-5,'TerminationMode',0,'OutputTermValidate',0,'OutputTermBuildCheck',0,'EnableEvent',0,'EventMode',1,'EventOnFalling',1,'EventOnRising',0,'EventDelay',0,'EventRate',1,'EventBuildCheck',0,'TriggerLine',1,'TLCFileName','rti120xdio_c1_pwm')
  DIO_CLASS1_PWM_BL8 : rti1202lib_dio_class1/DIO_CLASS1_PWM_BL1  Commented=on  DSProperties=struct('RTI',struct('Version',uint32(1),'BlockType',struct('isSLSource',uint8(0),'isSLSink',uint8(1),'isHWSource',uint8(0),'isHWSink',uint8(1),'isSetup',uint8(0),'isInline',uint8(1),'isNonInline',uint8(0),'isInterrupt',uint8(0),'isChannelwise',uint8(1)),'IOBoardType',{{'DS120X','STD','DIOC1'}},'UnitType','PWM','Identifier','PWM','DialogType','ML','BlockSet','NONE','SlaveProcessor','NONE'))  RTIBlockInterface=struct('InputPortsWidth',int32([1 1]),'InputPortsActive',[1 1],'InputPortsName',{{'Period',['Duty Cycle']}},'BlockDisplay',{{['DIO CL1 PWM\nPort: 1\nChannel: 3'],'center'}},'IconTransparency','on','InitLevel',3,'DialogFcn','rti120xstddioc1pwmgui','BlockName',struct('Token',{{'DIO_CLASS1_PWM_BL1'}}))  RTIBlockParameters=struct('PortNo',{{1,'OFF',[]}},'ChannelNo',{{3,'OFF',[]}},'HighLevel',{{3,'OFF',[1 3]}},'UpdateMode',{{1,'OFF',[1 2]}},'InvertingMode',{{1,'OFF',[1 2]}},'DutyCycleInit',{{'0.5','OFF',[0 1]}},'DutyCycleTerm',{{'0.5','OFF',[0 1]}},'PeriodInit',{{'5e-05','OFF',[1e-7 1.34]}},'PeriodTerm',{{'5e-05','OFF',[1e-7 1.34]}},'TerminationMode',{{0,'OFF',[0 1]}},'OutputTermValidate',{{0,'OFF',[0 1]}},'OutputTermBuildCheck',{{false,'OFF',[]}},'EnableEvent',{{0,'OFF',[0 1]}},'EventMode',{{1,'OFF',[1 3]}},'EventOnFalling',{{1,'OFF',[0 1]}},'EventOnRising',{{0,'OFF',[0 1]}},'EventDelay',{{'0','OFF',[0 1.34]}},'EventRate',{{'1','OFF',[1 256]}},'EventBuildCheck',{{false,'OFF',[]}},'TriggerLine',{{1,'OFF',[1 16]}},'TLCFileName',{{'rti120xdio_c1_pwm','OFF',[]}})  RTISFcnParameters=struct('PortNo','int16','ChannelNo','int16','HighLevel','int16','UpdateMode','int16','InvertingMode','int16','DutyCycleInit','double','DutyCycleTerm','double','PeriodInit','double','PeriodTerm','double','TerminationMode','int16','OutputTermValidate','int16','EnableEvent','int16','EventMode','int16','EventOnFalling','int16','EventOnRising','int16','EventDelay','double','EventRate','int16','TriggerLine','int16','TLCFileName','char')  RTIBlockParaDefault=struct('PortNo',1,'ChannelNo',1,'HighLevel',1,'UpdateMode',1,'InvertingMode',1,'DutyCycleInit',2^-1,'DutyCycleTerm',2^-1,'PeriodInit',5e-5,'PeriodTerm',5e-5,'TerminationMode',0,'OutputTermValidate',0,'OutputTermBuildCheck',0,'EnableEvent',0,'EventMode',1,'EventOnFalling',1,'EventOnRising',0,'EventDelay',0,'EventRate',1,'EventBuildCheck',0,'TriggerLine',1,'TLCFileName','rti120xdio_c1_pwm')
  DP_calc : Subsystem  Commented=on
  DP_ref : Scope
      settings: ActiveDisplayYMinimum=-27.57876  ActiveDisplayYMaximum=127.57876  DataLoggingVariableName=ScopeData2
  DTM_RPM : Scope  Commented=on
      settings: ActiveDisplayYMinimum=-0.19312  ActiveDisplayYMaximum=4.51012
  DTM_RPM1 : Scope  Commented=on
      settings: ActiveDisplayYMinimum=1000  ActiveDisplayYMaximum=11000
  DVAD : Constant  Commented=on  Value=50
  DV_calc : Subsystem  Commented=on
  D_1_Sp : Constant  Commented=on  Value=0.012
  Delta_P2_tank_atm_Pa1 : Scope
      settings: ActiveDisplayYMinimum=-477.29276  ActiveDisplayYMaximum=7335.37644  DataLoggingVariableName=ScopeData4
  Delta_P2_tank_atm_Pa2 : Scope
      settings: ActiveDisplayYMinimum=-477.29276  ActiveDisplayYMaximum=7335.37644  DataLoggingVariableName=ScopeData5
  Delta_P_compressor_Pa1 : Scope
      settings: ActiveDisplayYMinimum=465869.568  ActiveDisplayYMaximum=472095.7054  DataLoggingVariableName=ScopeData6
  Delta_P_tank_Pa1 : Scope
      settings: ActiveDisplayYMinimum=-477.29276  ActiveDisplayYMaximum=7335.37644  DataLoggingVariableName=ScopeData7
  Delta_P_tank_Pa2 : Scope
      settings: ActiveDisplayYMinimum=-477.29276  ActiveDisplayYMaximum=7335.37644  DataLoggingVariableName=ScopeData8
  Demux : Demux  Outputs=5
  Demux1 : Demux  Outputs=3
  Demux2 : Demux  Outputs=8
  Derivative3 : Derivative  Commented=on
  Derivative5 : Derivative  Commented=on
  Discrete-Time Integrator : DiscreteIntegrator  Commented=on  SampleTime=-1  ICPrevOutput=DiscIntNeverNeededParam  ICPrevScaledInput=DiscIntNeverNeededParam
  Display : Display  Commented=on
  Display1 : Display  Commented=on
  Divide{,1..4} (5 alike) : Product  Inputs=**
  Divide8 : Product  Commented=on  Inputs=*/
  Divide9 : Product  Commented=on  Inputs=**
  E2 : Scope
  Edge Detector1 : dspswit3/Edge Detector  Commented=on  InputProcessing=Columns as channels (frame based)
  Enable_pin : Constant  Commented=on  Value=0  OutDataTypeStr=boolean
  Error_ITM : Scope  Commented=on
  Fcn : Fcn  Commented=on  Expr=u*0.05 + 0.05
  From3 : From  Commented=on  GotoTag=Qvad_m3_s
  From34 : From  Commented=on  GotoTag=Qvad_kalman  TagVisibility=global
  From35 : From  Commented=on  GotoTag=ref_of_pwm
  From4 : From  Commented=on  GotoTag=SP_sw
  From67 : From  Commented=on  GotoTag=VAD_enable
  From73 : From  Commented=on  GotoTag=SP_l_min_raw  TagVisibility=global
  From74 : From  Commented=on  GotoTag=Qlvad_l_min_raw  TagVisibility=global
  From76 : From  Commented=on  GotoTag=Qsp_kalman  TagVisibility=global
  G2_PWM : Scope  Commented=on
      settings: DataLoggingVariableName=ScopeData10
  G3_PWM : Scope  Commented=on
      settings: DataLoggingVariableName=ScopeData11
  G4_PWM : Scope  Commented=on
      settings: DataLoggingVariableName=ScopeData12
  G5_PWM : Scope  Commented=on
      settings: DataLoggingVariableName=ScopeData13
  GP_KAPATT : Constant  Commented=on
  Gain{,3,7,17..18,20..23,26,30,32..33} (13 alike) : Gain  Gain=1/133.32
  Gain{8..10,28..29} (5 alike) : Gain  Gain=1e-6
  Gain{11..12,35..36} (4 alike) : Gain  Commented=on  Gain=1.6667e-5
  Gain13 : Gain  Commented=on  Gain=10
  Gain14 : Gain  Commented=on  Gain=1000
  Gain15 : Gain  Gain=133.32
  Gain16 : Gain  Gain=133.32
  Gain19 : Gain
  Gain2 : Gain  Commented=on  Gain=10
  Gain25 : Gain  Gain=1/16.6666
  Gain27 : Gain  Gain=1/16.6666
  Gain31 : Gain  Gain=133.32
  Gain34 : Gain  Gain=8
  Gain37 : Gain  Commented=on  Gain=1000
  Gain38 : Gain  Gain=1/1.6667e-5
  Gain39 : Gain  Gain=1/1.6667e-5
  Gain4 : Gain  Commented=on  Gain=10
  Gain40 : Gain  Commented=on  Gain=1/9620
  Gain41 : Gain  Gain=1/1.6667e-5
  Gain42 : Gain  Commented=on
  Gain6 : Gain  Commented=on  Gain=1000
  Goto12 : Goto  Commented=on  GotoTag=Qin_m3_s_raw  TagVisibility=global
  Goto13 : Goto  Commented=on  GotoTag=Qout_m3_s_raw  TagVisibility=global
  Goto22 : Goto  Commented=on  GotoTag=Qin_l_min_raw  TagVisibility=global
  Goto23 : Goto  Commented=on  GotoTag=Qout_l_min_raw  TagVisibility=global
  Goto3 : Goto  Commented=on  GotoTag=sp_PWM  TagVisibility=global
  Goto46 : Goto  Commented=on  GotoTag=gp_PWM  TagVisibility=global
  Goto47 : Goto  Commented=on  GotoTag=valve_switch  TagVisibility=global
  Goto48 : Goto  Commented=on  GotoTag=C_on_off  TagVisibility=global
  Goto49 : Goto
  Goto59 : Goto  Commented=on  GotoTag=Qlvad_l_min_raw  TagVisibility=global
  Goto60 : Goto  Commented=on  GotoTag=Qlvad_m3_s_raw  TagVisibility=global
  Goto61 : Goto  Commented=on  GotoTag=Qgp_l_min_raw  TagVisibility=global
  Goto62 : Goto  Commented=on  GotoTag=Qgp_m3_s_raw  TagVisibility=global
  Goto66 : Goto  Commented=on  GotoTag=SP_l_min_raw  TagVisibility=global
  Goto69 : Goto  Commented=on  GotoTag=SP_sw
  Goto70 : Goto  Commented=on  GotoTag=VAD_enable
  Goto73 : Goto  Commented=on  GotoTag=VADL  TagVisibility=global
  Goto74 : Goto  Commented=on  GotoTag=zort
  Goto76 : Goto  Commented=on  GotoTag=SP_m3_s_raw  TagVisibility=global
  IBS_LVAD : Subsystem  Commented=on
  "IBS_o " : Scope  Commented=on
      settings: DataLoggingVariableName=ScopeData2
  IVAD : Constant  Commented=on  Value=500
  I_1_Sp : Constant  Commented=on  Value=0.08
  Integrator4 : Integrator  Commented=on  ExternalReset=either
  Integrator7 : Integrator  Commented=on  ExternalReset=either  InitialCondition=1500
  K1 : Constant  Value=-50
  K2 : Constant  Value=-300
  K3 : Constant  Value=-100
  K4 : Constant  Value=-300
  K5 : Constant  Value=-500
  KALMAN 3 STATES PLA : Subsystem  Commented=on
  K_1_Sp : Constant  Commented=on  Value=0.8
  LVAD_BS : Scope  Commented=on
      settings: DataLoggingVariableName=ScopeData3
  LV_f_ow : Constant  Commented=on  Value=0
  LV_r_ow : Constant  Commented=on  Value=0
  LV_release_current : From  Commented=on  GotoTag=LV_release_input_Current  TagVisibility=global
  LV_tank_fill_current : From  Commented=on  GotoTag=LV_Fill_current  TagVisibility=global
  MATLAB Function2 : MATLAB Function  TreatAsAtomicUnit=on
  MATLAB Function4 : MATLAB Function  Commented=on  TreatAsAtomicUnit=on
  MATLAB Function5 : MATLAB Function  Commented=on  TreatAsAtomicUnit=on
  MATLAB Function6 : MATLAB Function  TreatAsAtomicUnit=on
  MATLAB Function7 : MATLAB Function  Commented=on  TreatAsAtomicUnit=on
  MATLAB Function8 : MATLAB Function  Commented=on  TreatAsAtomicUnit=on
  MATLAB Function9 : MATLAB Function  Commented=on  TreatAsAtomicUnit=on
  Motor PWM : Constant  Commented=on  Value=0
  Motor PWM Period : Constant  Commented=on  Value=0.02
  Motor_PWM : Scope  Commented=on
      settings: ActiveDisplayYMinimum=-1  ActiveDisplayYMaximum=1
  Motor_PWM1 : Scope  Commented=on
      settings: DataLoggingVariableName=ScopeData2
  Motor_RPM_Override : Constant  Commented=on  Value=0
  Moving Average : dspstat3/Moving Average  Commented=on  Method=Sliding window  ForgettingFactorPort=off  SpecifyWindowLength=on  WindowLengthSource=Property  MaxWindowLength=20  WindowLength=100  OverlapLength=99  AllowArbitraryInputLength=off  ForgettingFactor=0.9  SimulateUsing=Code generation
  Moving Average1 : dspstat3/Moving Average  Commented=on  Method=Sliding window  ForgettingFactorPort=off  SpecifyWindowLength=on  WindowLengthSource=Property  MaxWindowLength=20  WindowLength=100  OverlapLength=99  AllowArbitraryInputLength=off  ForgettingFactor=0.9  SimulateUsing=Code generation
  Mux : Mux  Inputs=8
  Mux1 : Mux  Inputs=5
  Mux2 : Mux  Inputs=8
  Mux3 : Mux  Inputs=3
  Mux4 : Mux  Inputs=8
  ON_OF_SP : Constant  Commented=on  Value=0
  P1 : ZeroOrderHold  SampleTime=dt_k
  P1_Pa_raw : Scope
      settings: ActiveDisplayYMinimum=-70.75678  ActiveDisplayYMaximum=637.64659
  P1_mmHg_kalman : Scope
      settings: ActiveDisplayYMinimum=-1.1884374265645462E+299  ActiveDisplayYMaximum=1.3204860295161621E+298  DataLoggingVariableName=ScopeData18
  P1_mmHg_raw : Scope
      settings: ActiveDisplayYMinimum=-70.75678  ActiveDisplayYMaximum=637.64659  DataLoggingVariableName=ScopeData2
  P1_ref : Constant  Value=P1refmmHg
  P1_ref_mmhg : Scope
      settings: DataLoggingVariableName=ScopeData20
  P1ref : ZeroOrderHold  SampleTime=dt_k
  P2 : ZeroOrderHold  SampleTime=dt_k
  P2 Fill : MATLAB Function  TreatAsAtomicUnit=on
  P2 Release : MATLAB Function  TreatAsAtomicUnit=on
  P2_Pa_kalman : Scope
      settings: ActiveDisplayYMinimum=-0.09224  ActiveDisplayYMaximum=0.83329
  P2_Pa_raw : Scope
      settings: ActiveDisplayYMinimum=-70.75678  ActiveDisplayYMaximum=637.64659  DataLoggingVariableName=ScopeData22
  P2_mmHg_kalman : Scope
      settings: ActiveDisplayYMinimum=-0.09224  ActiveDisplayYMaximum=0.83329  DataLoggingVariableName=ScopeData23
  P2_mmHg_raw : Scope
      settings: ActiveDisplayYMinimum=-70.75678  ActiveDisplayYMaximum=637.64659  DataLoggingVariableName=ScopeData24
  P2_p : ZeroOrderHold  SampleTime=dt_k
  P2_p_mmHg_raw : Scope
      settings: ActiveDisplayYMinimum=-70.75678  ActiveDisplayYMaximum=637.64659  DataLoggingVariableName=ScopeData25
  P2_ref_mmhg : Scope
      settings: ActiveDisplayYMinimum=99.6823  ActiveDisplayYMaximum=160.3177  DataLoggingVariableName=ScopeData26
  P2_sin1 : Sin  Amplitude=0  Bias=55  Frequency=8  SampleTime=0
  P2_sin2 : Sin  Amplitude=0  Frequency=13  Phase=4  SampleTime=0
  P2p_Pa_raw : Scope
      settings: ActiveDisplayYMinimum=-70.75678  ActiveDisplayYMaximum=637.64659  DataLoggingVariableName=ScopeData2
  P2p_mmHg_kalman : Scope
      settings: ActiveDisplayYMinimum=-5.0502138038964361E+156  ActiveDisplayYMaximum=4.5451924235067935E+157  DataLoggingVariableName=ScopeData28
  P2ref : ZeroOrderHold  SampleTime=dt_k
  P3 : ZeroOrderHold  SampleTime=dt_k
  P3 Fill : MATLAB Function  TreatAsAtomicUnit=on
  P3 Release : MATLAB Function  TreatAsAtomicUnit=on
  P3_Pa_kalman : Scope
      settings: ActiveDisplayYMinimum=-0.09224  ActiveDisplayYMaximum=0.83329  DataLoggingVariableName=ScopeData2
  P3_Pa_raw : Scope
      settings: ActiveDisplayYMinimum=-70.75678  ActiveDisplayYMaximum=637.64659  DataLoggingVariableName=ScopeData30
  P3_mmHg_kalman : Scope
      settings: ActiveDisplayYMinimum=-4.523595627601701E+157  ActiveDisplayYMaximum=5.0262173640018894E+156  DataLoggingVariableName=ScopeData31
  P3_mmHg_raw : Scope
      settings: ActiveDisplayYMinimum=-70.75678  ActiveDisplayYMaximum=637.64659  DataLoggingVariableName=ScopeData32
  P3_p : ZeroOrderHold  SampleTime=dt_k
  P3_p_mmHg_raw : Scope
      settings: ActiveDisplayYMinimum=-70.75678  ActiveDisplayYMaximum=637.64659  DataLoggingVariableName=ScopeData33
  P3_ref_mmhg : Scope
      settings: ActiveDisplayYMinimum=20  ActiveDisplayYMaximum=40  DataLoggingVariableName=ScopeData34
  P3_sin1 : Sin  Amplitude=0  Bias=40  Frequency=7  Phase=5  SampleTime=0
  P3_sin2 : Sin  Amplitude=0  Frequency=19  Phase=15
  P3p_Pa_raw : Scope
      settings: ActiveDisplayYMinimum=-70.75678  ActiveDisplayYMaximum=637.64659  DataLoggingVariableName=ScopeData35
  P3p_mmHg_kalman : Scope
      settings: ActiveDisplayYMinimum=-4.6199274720354334E+157  ActiveDisplayYMaximum=5.1332527467060366E+156  DataLoggingVariableName=ScopeData36
  P3ref : ZeroOrderHold  SampleTime=dt_k
  PID Controller : slpidlib/PID Controller  Commented=on  Controller=PID  Form=Parallel  TimeDomain=Continuous-time  UseExternalTs=off  SampleTime=-1  IntegratorMethod=Forward Euler  FilterMethod=Forward Euler  ControllerParametersSource=external  P=1  I=1  UseKiTs=off  D=0  UseExternalDerivativeSource=off  N=100  UseFilter=on  TunerSelectOption=Transfer Function Based (PID Tuner App)  InitialConditionSource=internal  InitialConditionForIntegrator=0  InitialConditionForFilter=0  DifferentiatorICPrevScaledInput=0  ExternalReset=none  TrackingMode=off  Kt=1  LimitOutput=off  SatLimitsSource=internal  UpperSaturationLimit=inf  LowerSaturationLimit=-inf  LinearizeAsGain=on  AntiWindupMode=none  Kb=1  LimitIntegrator=off  UpperIntegratorSaturationLimit=inf  LowerIntegratorSaturationLimit=-inf  POutMin=[]  POutMax=[]  IOutMin=[]  IOutMax=[]  DOutMin=[]  DOutMax=[]  NOutMin=[]  NOutMax=[]  SumOutMin=[]  SumOutMax=[]  SaturationOutMin=[]  SaturationOutMax=[]  PParamMin=[]  PParamMax=[]  IParamMin=[]  IParamMax=[]  DParamMin=[]  DParamMax=[]  NParamMin=[]  NParamMax=[]  KbParamMin=[]  KbParamMax=[]  KtParamMin=[]  KtParamMax=[]  KbOutMin=[]  KbOutMax=[]  KtOutMin=[]  KtOutMax=[]  IntegratorOutMin=[]  IntegratorOutMax=[]  FilterOutMin=[]  FilterOutMax=[]  SumI1OutMin=[]  SumI1OutMax=[]  SumI2OutMin=[]  SumI2OutMax=[]  SumI3OutMin=[]  SumI3OutMax=[]  SumI4OutMin=[]  SumI4OutMax=[]  SumDOutMin=[]  SumDOutMax=[]  DifferentiatorOutMin=[]  DifferentiatorOutMax=[]  FilterDiffOutCoefMin=[]  FilterDiffOutCoefMax=[]  ReciprocalOutMin=[]  ReciprocalOutMax=[]  SumDenOutMin=[]  SumDenOutMax=[]  SumNumOutMin=[]  SumNumOutMax=[]  DivideOutMin=[]  DivideOutMax=[]  UdiffTsProdOutMin=[]  UdiffTsProdOutMax=[]  NTsProdOutMin=[]  NTsProdOutMax=[]  UintegralTsProdOutMin=[]  UintegralTsProdOutMax=[]  UngainTsProdOutMin=[]  UngainTsProdOutMax=[]  ClampingZeroOutDataTypeStr=Inherit: Inherit via back propagation  ClampingZeroOutMin=[]  ClampingZeroOutMax=[]  FilterDenConstantOutDataTypeStr=Inherit: Inherit via back propagation  FilterDenConstantOutMin=[]  FilterDenConstantOutMax=[]  PCopyOutDataTypeStr=Inherit: Inherit via back propagation  PCopyOutMin=[]  PCopyOutMax=[]  NCopyOutDataTypeStr=Inherit: Inherit via back propagation  NCopyOutMin=[]  NCopyOutMax=[]  IntegratorContinuousStateAttributes=''  IntegratorStateMustResolveToSignalObject=off  IntegratorRTWStateStorageClass=Auto  FilterContinuousStateAttributes=''  FilterStateMustResolveToSignalObject=off  FilterRTWStateStorageClass=Auto  ParallelPVariant=ExternalParameters  IdealPVariant=Disabled  IVariant=ExternalParameters  DVariant=ExternalParameters  IntegratorVariant=Continuous  SatVariant=Disabled  AWVariant=Passthrough  PCopyVariant=Disabled  TRVariant=Disabled  FdbkBlocksVariant=Forward  IdealPFdbkVariant=Disabled  SatFdbkVariant=Disabled  DerivativeFilterVariant=ContFilter  NVariant=ExternalParameters  NCopyVariant=Disabled  FilterICVariant=InternalICsFilter  IntegratorICVariant=InternalICs  ExternalResetVariant=Disabled  TRSumVariant=Passthrough  SumFdbkVariant=Disabled  SumVariant=Sum_PID  TsampFilterVariant=InternalTs  TsampNgainVariant=Passthrough  TsampIntegralVariant=Disabled_SignalSpec  ExternalSaturationOutDataTypeStr=Inherit: Same as second input  DerivativeSourceVariant=ErrorSignal  PreIntVariant=InternalPreInt
  PID_of_D : Gain  Commented=on  Gain=0.001
  PID_of_I : Gain  Commented=on  Gain=0.001
  PID_of_P : Gain  Commented=on  Gain=0.001
  PID_of_PID_ITM : Constant  Commented=on  Value=0
  PVAD : Constant  Commented=on  Value=8000
  PVac : ZeroOrderHold  SampleTime=dt_k
  PWM Period1 : Constant  Commented=on  Value=PWM_Period_g2
  PWM Period2 : Constant  Commented=on  Value=PWM_Period_g3
  PWM Period3 : Constant  Commented=on  Value=PWM_Period_g4
  PWM Period4 : Constant  Commented=on  Value=PWM_Period_g5
  PWM Period5 : Constant  Commented=on  Value=PWM_Period
  PWM Period6 : Constant  Commented=on  Value=PWM_Period
  "P_Vac_mmHg " : Scope
      settings: DataLoggingVariableName=ScopeData37
  Pc : ZeroOrderHold  SampleTime=dt_k
  Pcomp_Pa_raw : Scope
      settings: ActiveDisplayYMinimum=-70.75678  ActiveDisplayYMaximum=637.64659  DataLoggingVariableName=ScopeData38
  Pcomp_mmHg : Scope
      settings: ActiveDisplayYMinimum=-70.75678  ActiveDisplayYMaximum=637.64659  DataLoggingVariableName=ScopeData39
  Pin_mmHg_kalman : Scope
      settings: DataLoggingVariableName=ScopeData40
  Pin_mmHg_raw : Scope
      settings: ActiveDisplayYMinimum=-70.75678  ActiveDisplayYMaximum=637.64659  DataLoggingVariableName=ScopeData41
  "Pkalman " : Scope
      settings: ActiveDisplayYMinimum=0.00883  ActiveDisplayYMaximum=0.02957  DataLoggingVariableName=ScopeData42
  Pout_mmHg_kalman : Scope
      settings: ActiveDisplayYMinimum=-0.09224  ActiveDisplayYMaximum=0.83329  DataLoggingVariableName=ScopeData43
  Pout_mmHg_raw : Scope
      settings: ActiveDisplayYMinimum=-1  ActiveDisplayYMaximum=1  DataLoggingVariableName=ScopeData44
  Product{,2..16,20} (17 alike) : Product  Commented=on
  Pvac_Pa_raw1 : Scope
      settings: ActiveDisplayYMinimum=-70.75678  ActiveDisplayYMaximum=637.64659  DataLoggingVariableName=ScopeData3
  Pvac_mmHg : Scope
      settings: ActiveDisplayYMinimum=-70.75678  ActiveDisplayYMaximum=637.64659  DataLoggingVariableName=ScopeData46
  Q{1..5} (5 alike) : Scope
      Q1 settings: ActiveDisplayYMinimum=-13.75  ActiveDisplayYMaximum=123.75  DataLoggingVariableName=ScopeData47
      Q2 settings: ActiveDisplayYMinimum=-8.75  ActiveDisplayYMaximum=78.75  DataLoggingVariableName=ScopeData48
      Q3 settings: ActiveDisplayYMinimum=-1  ActiveDisplayYMaximum=1  DataLoggingVariableName=ScopeData49
      Q4 settings: ActiveDisplayYMinimum=-8.75  ActiveDisplayYMaximum=78.75  DataLoggingVariableName=ScopeData50
      Q5 settings: ActiveDisplayYMinimum=-1  ActiveDisplayYMaximum=1  DataLoggingVariableName=ScopeData51
  Q_Sys_std : Constant  Value=Q_Sys_std
  Q_gp : ZeroOrderHold  SampleTime=dt_k
  Q_sp : ZeroOrderHold  SampleTime=dt_k
  Q_vad : ZeroOrderHold  SampleTime=dt_k
  Qgp_l_min_kalman : Scope
      settings: ActiveDisplayYMinimum=-3.3540427399502875E+162  ActiveDisplayYMaximum=3.0186384659552592E+163  DataLoggingVariableName=ScopeData55
  Qgp_l_min_raw : Scope  Commented=on
      settings: ActiveDisplayYMinimum=539.53184  ActiveDisplayYMaximum=1116.19693  DataLoggingVariableName=ScopeData56
  Qgp_m3_s_kalman : Scope
      settings: ActiveDisplayYMinimum=-3.3540427399502875E+162  ActiveDisplayYMaximum=3.0186384659552592E+163  DataLoggingVariableName=ScopeData3
  Qgp_m3_s_raw : Scope  Commented=on
      settings: ActiveDisplayYMinimum=539.53184  ActiveDisplayYMaximum=1116.19693  DataLoggingVariableName=ScopeData57
  Qgp_ml_min_raw : Scope  Commented=on
      settings: ActiveDisplayYMinimum=539.53184  ActiveDisplayYMaximum=1116.19693  DataLoggingVariableName=ScopeData58
  Qin : ZeroOrderHold  SampleTime=dt_k
  Qk_Gain_P1 : Constant  Value=1e-6
  Qk_Gain_P2 : Constant  Value=1e-6
  Qk_Gain_P2p : Constant  Value=1e-6
  Qk_Gain_P3 : Constant  Value=1e-6
  Qk_Gain_P3p : Constant  Value=1e-6
  Qk_Gain_Qgp : Constant  Value=1e-6
  Qk_Gain_Qvad : Constant  Value=1e-6
  Qk_Gain_Qvad1 : Constant  Value=1e-6
  Qlvad_l_min_raw : Scope  Commented=on
      settings: ActiveDisplayYMinimum=539.53184  ActiveDisplayYMaximum=1116.19693  DataLoggingVariableName=ScopeData59
  Qlvad_m3_s_raw : Scope  Commented=on
      settings: ActiveDisplayYMinimum=539.53184  ActiveDisplayYMaximum=1116.19693  DataLoggingVariableName=ScopeData60
  Qlvad_ml_min_raw : Scope  Commented=on
      settings: ActiveDisplayYMinimum=539.53184  ActiveDisplayYMaximum=1116.19693  DataLoggingVariableName=ScopeData61
  Qout : ZeroOrderHold  SampleTime=dt_k
  Qsp_l_min_kalman : Scope
      settings: ActiveDisplayYMinimum=-3.3540427399502875E+162  ActiveDisplayYMaximum=3.0186384659552592E+163
  Qsp_l_min_raw : Scope  Commented=on
      settings: ActiveDisplayYMinimum=539.53184  ActiveDisplayYMaximum=1116.19693
  Qsp_m3_s_raw : Scope  Commented=on
      settings: ActiveDisplayYMinimum=539.53184  ActiveDisplayYMaximum=1116.19693  DataLoggingVariableName=ScopeData2
  Qsp_ml_min_raw : Scope  Commented=on
      settings: ActiveDisplayYMinimum=539.53184  ActiveDisplayYMaximum=1116.19693  DataLoggingVariableName=ScopeData3
  Qvad_l_min_kalman1 : Scope
      settings: ActiveDisplayYMinimum=-0.08507  ActiveDisplayYMaximum=-0.03736  DataLoggingVariableName=ScopeData63
  Qvad_m3_s_kalman : Scope
      settings: ActiveDisplayYMinimum=-3.3540427399502875E+162  ActiveDisplayYMaximum=3.0186384659552592E+163  DataLoggingVariableName=ScopeData4
  RPM_read : Scope  Commented=on
      settings: ActiveDisplayYMinimum=-188162.82273  ActiveDisplayYMaximum=1.964541577E+6
  RPM_read2 : Scope  Commented=on
      settings: ActiveDisplayYMinimum=-188162.82273  ActiveDisplayYMaximum=1.964541577E+6  DataLoggingVariableName=ScopeData2
  RTI Data : Subsystem  Tag=struct('RTIDataServer',struct('RTIDataServerVs','2','RTIModelDescription','struct(''main'',''HMC'',''sub'',''HMC'',''isMp'',0)'))  LoadFcn="if exist('rtidc'), try,  rtidc('DataHostBlockClbLoad', gcbh); catch, disp(['Warning: ''LoadFcn'' for RTI Data block failed: ' lasterr]); end, end,"  mask(RTI_DATA_HOST){}
      mask help:
      | RTI Data Block.
      | This block is used by RTI to store internal model-dependent data.
      | Please keep this block on the root level of the model. Deleting this block will result in data loss.
      |
      | NEVER DELETE OR COPY THIS BLOCK!
      settings: CopyFcn="if exist('rtidc'), try,  rtidc('DataHostBlockClbCopy', gcbh); catch, disp(['Warning: ''CopyFcn'' for RTI Data block failed: ' lasterr]); end, end,"  DeleteFcn="if exist('rtidc'), try,  rtidc('DataHostBlockClbDelete', gcbh); catch, disp(['Warning: ''DeleteFcn'' for RTI Data block failed: ' lasterr]); end, end,"  ModelCloseFcn="if exist('rtidc'), try,  rtidc('DataHostBlockClbModelClose', gcbh); catch, disp(['Warning: ''ModelCloseFcn'' for RTI Data block failed: ' lasterr]); end, end,"  PreSaveFcn="if exist('rtidc'), try,  rtidc('DataHostBlockClbPreSave', gcbh); catch, disp(['Warning: ''PreSaveFcn'' for RTI Data block failed: ' lasterr]); end, end,"  PostSaveFcn="if exist('rtidc'), try,  rtidc('DataHostBlockClbPostSave', gcbh); catch, disp(['Warning: ''PostSaveFcn'' for RTI Data block failed: ' lasterr]); end, end,"  NameChangeFcn="if exist('rtidc'), try,  rtidc('DataHostBlockClbNameChange', gcbh); catch, disp(['Warning: ''NameChangeFcn'' for RTI Data block failed: ' lasterr]); end, end,"
      mask Help:
      | RTI Data Block.
      | This block is used by RTI to store internal model-dependent data.
      | Please keep this block on the root level of the model. Deleting this block will result in data loss.
      | 
      | NEVER DELETE OR COPY THIS BLOCK!
      mask Display:
      | text(0.5, 0.5, 'RTI Data', 'HorizontalAlignment', 'center');
      | plot([1 0]);
  R_Meas_std : Constant  Value=R_Meas_std
  Real_IBS : Subsystem  Commented=on
  Reference CVSs : Subsystem
  Relational Operator : RelationalOperator  Commented=on  OutDataTypeStr=boolean  RndMeth=Simplest  InputSameDT=off
  Rk_Gain_P1 : Constant  Value=1e-4
  Rk_Gain_P2 : Constant  Value=1e-4
  Rk_Gain_P2p : Constant  Value=1e-4
  Rk_Gain_P3 : Constant  Value=1e-4
  Rk_Gain_P3p : Constant  Value=1e-4
  Rk_Gain_Qgp : Constant  Value=7.5173e-4
  Rk_Gain_Qsp : Constant  Value=6.3571e-4
  Rk_Gain_Qvad : Constant  Value=6.3571e-4
  SP_pwm_override : Constant  Commented=on  Value=0
  Saturation{,1..2,12..13} (5 alike) : Saturate  UpperLimit=inf  LowerLimit=0
  Saturation{5..7,10..11} (5 alike) : Saturate  UpperLimit=200  LowerLimit=0
  Saturation16 : Saturate  Commented=on  UpperLimit=0.1  LowerLimit=0
  Saturation17 : Saturate  Commented=on  UpperLimit=0.99  LowerLimit=0
  Saturation18 : Saturate  Commented=on  UpperLimit=1  LowerLimit=0
  Saturation19 : Saturate  Commented=on  UpperLimit=1  LowerLimit=0
  Saturation20 : Saturate  Commented=on  UpperLimit=10  LowerLimit=-10
  Saturation3 : Saturate  Commented=on  UpperLimit=10  LowerLimit=-10
  Saturation4 : Saturate  Commented=on  UpperLimit=10  LowerLimit=-10
  Saturation8 : Saturate  Commented=on  UpperLimit=10000  LowerLimit=2000
  Saturation9 : Saturate  Commented=on  UpperLimit=1  LowerLimit=0
  Scope : Scope  NumInputPorts=2
      settings: DataLoggingVariableName=ScopeData4
  Scope{1..3,14} (4 alike) : Scope  Commented=on
      Scope14 settings: ActiveDisplayYMinimum=-0.15624  ActiveDisplayYMaximum=1.40614  DataLoggingVariableName=ScopeData4
      Scope2 settings: ActiveDisplayYMinimum=-0.19312  ActiveDisplayYMaximum=4.51012  DataLoggingVariableName=ScopeData2
      Scope3 settings: ActiveDisplayYMinimum=-0.125  ActiveDisplayYMaximum=1.125  DataLoggingVariableName=ScopeData3
  Small_Pump_Ref : Constant  Commented=on
  Subsystem : Subsystem  Commented=on
  Subsystem1 : Subsystem  Commented=on
  Subtract2 : Sum  Inputs=+-
  Sum{,1,3..5,7,18} (7 alike) : Sum  Commented=on  Inputs=|++
  Sum17 : Sum  Commented=on  Inputs=|+-
  Sum2 : Sum  Commented=on  Inputs=|+-
  Sum6 : Sum  Commented=on  Inputs=|+-
  Switch : Switch  Threshold=1  SaturateOnIntegerOverflow=off  InputSameDT=off
  Switch1 : Switch  Threshold=1  SaturateOnIntegerOverflow=off  InputSameDT=off
  Switch2 : Switch  Commented=on  Criteria=u2 > Threshold  SaturateOnIntegerOverflow=off  InputSameDT=off
  Switch7 : Switch  Commented=on  Criteria=u2 > Threshold  SaturateOnIntegerOverflow=off  InputSameDT=off
  Transfer Fcn : TransferFcn  Denominator=[10 1]
  Transfer Fcn1 : TransferFcn  Denominator=[10 1]
  Unit Delay : UnitDelay  SampleTime=-1
  Unit Delay1 : UnitDelay  SampleTime=-1
  Unit Delay10 : UnitDelay  InitialCondition=1e-3  SampleTime=dt_k
  Unit Delay14 : UnitDelay  InitialCondition=1e-3  SampleTime=dt_k
  Unit Delay2 : UnitDelay  Commented=on  SampleTime=-1
  Unit Delay3 : UnitDelay  InitialCondition=y_kalman_ini  SampleTime=dt_k
  Unit Delay4 : UnitDelay  InitialCondition=[P1refmmHg*133.32;P2_ref_bias*133.32;P3_ref_bias*133.32]  SampleTime=dt_k
  Unit Delay5 : UnitDelay  InitialCondition=P_kalman_ini  SampleTime=dt_k
  Unit Delay6 : UnitDelay  Commented=on  SampleTime=-1
  Unit Delay9 : UnitDelay  InitialCondition=1e-3  SampleTime=dt_k
  Upper Limit of Q = 110 : Saturate  UpperLimit=110  LowerLimit=0
  Upper Limit of Q = 70 : Saturate  UpperLimit=70  LowerLimit=0
  Upper Limit of Q = 70 1 : Saturate  UpperLimit=70  LowerLimit=0
  "Upper Limit of Q = 70 _2 " : Saturate  UpperLimit=70  LowerLimit=0
  Upper Limit of Q = 70 _2 1 : Saturate  UpperLimit=70  LowerLimit=0
  VAD_PID_ON_OFF : Constant  Commented=on  Value=0
  VAD_ref_Q : Constant  Commented=on  Value=0
  Vacuum Bias : Bias  Bias=-1  SaturateOnIntegerOverflow=off
  Valve_on_off : Constant  Commented=on  Value=0
  dt_k : Constant  Value=dt_k  VectorParams1D=off
  ed_de1 : Scope  Commented=on
      settings: ActiveDisplayYMinimum=-0.125  ActiveDisplayYMaximum=1.125  DataLoggingVariableName=ScopeData5
  edge_de : Scope  Commented=on
      settings: ActiveDisplayYMinimum=-1  ActiveDisplayYMaximum=1  DataLoggingVariableName=ScopeData6
  g{1..5} (5 alike) : Scope
      g1 settings: ActiveDisplayYMinimum=-1  ActiveDisplayYMaximum=1  DataLoggingVariableName=ScopeData77
      g2 settings: ActiveDisplayYMinimum=-1  ActiveDisplayYMaximum=1  DataLoggingVariableName=ScopeData79
      g3 settings: DataLoggingVariableName=ScopeData81
      g4 settings: ActiveDisplayYMinimum=-9E-5  ActiveDisplayYMaximum=0.00083  DataLoggingVariableName=ScopeData83
      g5 settings: DataLoggingVariableName=ScopeData85
  g2_current : Scope  Commented=on
      settings: ActiveDisplayYMinimum=-20.75  ActiveDisplayYMaximum=186.75  DataLoggingVariableName=ScopeData80
  g3_current : Scope  Commented=on
      settings: DataLoggingVariableName=ScopeData82
  g4_current : Scope  Commented=on
      settings: DataLoggingVariableName=ScopeData84
  g5_current : Scope  Commented=on
      settings: DataLoggingVariableName=ScopeData86
  gp_on_off : Constant  Commented=on  Value=0
  gp_pwm_override : Constant  Commented=on  Value=0
  m3/sec to l/min{,1..4} (5 alike) : Fcn  Expr="60000 *  u(1)"
  per : Scope  Commented=on
      settings: ActiveDisplayYMinimum=34.10541  ActiveDisplayYMaximum=46.58829
  pwm_scope : Scope  Commented=on
      settings: ActiveDisplayYMinimum=-1  ActiveDisplayYMaximum=1  DataLoggingVariableName=ScopeData88
  raw_rpm : Scope  Commented=on
      settings: ActiveDisplayYMinimum=-1  ActiveDisplayYMaximum=1  DataLoggingVariableName=ScopeData7
  ref_of_ITM : Constant  Commented=on  Value=0
  "ref_sp " : Scope  Commented=on
      settings: DataLoggingVariableName=ScopeData90
  rpm_mov_per : Scope  Commented=on
      settings: ActiveDisplayYMinimum=29.70639  ActiveDisplayYMaximum=32.65151  DataLoggingVariableName=ScopeData3
  sat{2..5} (4 alike) : Saturate  Commented=on  UpperLimit=0.99  LowerLimit=0
  small_pump_PWM : Scope  Commented=on
      settings: ActiveDisplayYMinimum=-1  ActiveDisplayYMaximum=1  DataLoggingVariableName=ScopeData91
  tag scope: Air_Tank_Fill_Current=global, Ao_Fill_current=global, Ao_release_input_Current=global, Delta_P1_P2_Pa=global, Delta_P1_P3_Pa=global, Delta_P2_Patm_Pa=global, Delta_P3_Patm_Pa=global, Delta_Pc_P1_Pa=global, E1=global, E2=global, E3=global, LV_Fill_current=global, LV_release_input_Current=global, P1_Pa=global, P1_Pa_raw=global, P2_Pa=global, P2_Pa_raw=global, P2_mmHg=global, P2_mmHg_raw=global, P2p_Pa=global, P2p_Pa_raw=global, P2p_mmHg=global, P2p_mmHg_raw=global, P3_Pa=global, P3_Pa_raw=global, P3_mmHg=global, P3_mmHg_raw=global, P3p_Pa=global, P3p_Pa_raw=global, P3p_mmHg=global, P3p_mmHg_raw=global, P_Vac_Pa=global, P_kalman=global, Pc_Pa=global, Pin_mmHg=global, Pin_mmHg_raw=global, Pout_mmHg=global, Pout_mmHg_raw=global, Q_P1_Tank_Fill=global, Q_PAo_Fill=global, Q_PAo_Release=global, Q_PLV_Fill=global, Q_PLV_Release=global, Qgp_kalman=global, Qgp_m3_s=global, Qk=global, Qsp_kalman=global, Qvad_kalman=global, Rk=global, g1=global, g2=global, g3=global, g4=global, g5=global, y_kalman=global
  wires:
  sat4/1 -> Product6/1
  [P1_Pa_raw] -> P1/1
  Gain33/1 -> "P_Vac_mmHg "/1
  Divide/1 -> m3/sec to l/min/1
  Gain38/1 -> [Qgp_kalman], Qgp_l_min_kalman/1
  [g2] -> Divide1/1
  P2 Release/1(input_Current) -> Saturation7/1
  [P_Vac_Pa] -> Gain33/1
  Rk_Gain_P3/1 -> Mux4/4
  MATLAB Function6/2(Rk) -> [Rk]
  Saturation7/1 -> [Ao_release_input_Current]
  Gain21/1 -> P3_mmHg_kalman/1, [P3_mmHg], Pin_mmHg_kalman/1, [Pin_mmHg]
  Mux4/1 -> MATLAB Function6/2(Rk_gain)
  "Upper Limit of Q = 70 _2 "/1 -> Q2/1, [Q_PAo_Fill]
  Qk_Gain_P2p/1 -> Mux/2
  Valve_on_off/1 -> Saturation9/1
  Mux/1 -> MATLAB Function6/1(Qk_gain)
  Ao_release_current/1 -> MATLAB Function5/1(u), g3_current/1  "mA"
  Unit Delay3/1 -> MATLAB Function2/1(y_kalman_in)
  Gain16/1 -> Scope/1, P2ref/1
  MATLAB Function6/1(Qk) -> [Qk]
  Constant3/1 -> P3 Fill/4(difference)
  Upper Limit of Q = 70 _2 1/1 -> [Q_PLV_Fill], Q4/1
  Upper Limit of Q = 70/1 -> Q3/1, [Q_PAo_Release]
  Rk_Gain_P2/1 -> Mux4/3
  [Qgp_m3_s] -> Qgp_m3_s_kalman/1, Gain38/1
  K1/1 -> Mux1/1
  Constant1/1 -> Compressor to P1 Fill/4(difference)
  [E2] -> E2/1, P2 Release/1(error)
  Bar2Pa5/1 -> Bias8/1  "P1p_Pa"
  [valve_switch] -> MATLAB Function2/16(VS)
  Bar2Pa3/1 -> Bias9/1  "P2p_Pa"
  Product8/1 -> Add15/1
  [Delta_P2_Patm_Pa] -> Gain8/1  "pascal"
  Demux2/2 -> [P2p_Pa]
  [Delta_Pc_P1_Pa] -> Divide/2
  [P3p_Pa] -> Add2/2  "pascal"
  P1_ref/1 -> Gain15/1, P1_ref_mmhg/1
  [E1] -> Compressor to P1 Fill/1(error)
  [P2p_Pa] -> Add5/2  "pascal"
  Gain3/1 -> P2_mmHg_raw/1, Pout_mmHg_raw/1, [Pout_mmHg_raw], [P2_mmHg_raw]
  sat5/1 -> Product7/1
  MATLAB Function5/1(y) -> sat3/1  "duty_G3"
  P3/1 -> Mux2/4
  m3/sec to l/min3/1 -> Upper Limit of Q = 70 1/1  "Q_opt_tank"
  Saturation17/1 -> DIO_CLASS1_PWM_BL6/2, pwm_scope/1, Goto46/1
  Upper Limit of Q = 70 1/1 -> [Q_PLV_Release], Q5/1
  Saturation18/1 -> Scope3/1, DAC_CLASS1_BL1/1
  [g4] -> Divide3/1
  [P1_Pa] -> Add2/1  "pascal"
  [Q_PAo_Fill] -> P2 Fill/3(Q_Calculated)
  [Delta_P1_P2_Pa] -> Divide1/2
  Add21/1 -> Product9/1
  m3/sec to l/min1/1 -> Upper Limit of Q = 70/1  "Q_opt_tank"
  [P3_Pa] -> P3_Pa_kalman/1, Gain21/1
  Product15/1 -> sat4/1
  Demux/2 -> Saturation1/1
  Gain13/1 -> Bias4/1
  Add12/1 -> Switch1/1
  Unit Delay9/1 -> MATLAB Function2/15(kalman_z2)
  Constant15/1 -> Add12/2, Add11/1
  Product4/1 -> Add15/2
  Qk_Gain_P2/1 -> Mux/3
  [g1] -> Divide/1
  ADC_CLASS1_BL4/1 -> Bar2Pa3/1  "Analog Ch 4"
  Divide3/1 -> m3/sec to l/min4/1
  [P2p_Pa] -> Add6/1  "pascal"
  Demux2/6 -> [Qgp_m3_s]
  [E3] -> P3 Release/1(error)
  Constant6/1 -> P3 Release/4(difference)
  Gain28/1 -> P3 Fill/2(Measured_Delta_P)  "MPa"
  P2_sin2/1 -> Add/2
  [P2p_Pa] -> Gain22/1
  Q_vad/1 -> Mux2/7
  P3 Release/1(input_Current) -> Saturation11/1
  Gain18/1 -> Pcomp_mmHg/1
  [P3_Pa_raw] -> P3/1
  MATLAB Function2/4(Er) -> Demux1/1
  Unit Delay5/1 -> MATLAB Function2/2(P_kalman_in)
  [Delta_P1_P3_Pa] -> Gain28/1  "pascal"
  Add11/1 -> Switch/1
  dt_k/1 -> MATLAB Function2/10(dt)
  Gain12/1 -> Goto13/1, Qgp_m3_s_raw/1, Goto62/1
  [Qk] -> MATLAB Function2/3(Qk)
  Q_gp/1 -> Mux2/6
  P3 Fill/1(input_Current) -> Saturation10/1
  Switch/1 -> Subtract2/1, [P2_ref_mmHg], Gain16/1, P2_ref_mmhg/1
  Saturation19/1 -> DIO_CLASS1_PWM_BL8/2, Goto3/1, small_pump_PWM/1
  Rk_Gain_P2p/1 -> Mux4/2
  Saturation12/1 -> g4/1, [g4]
  [Qvad_m3_s] -> Qvad_m3_s_kalman/1, Gain39/1
  m3/sec to l/min/1 -> Upper Limit of Q = 110/1  "Q_opt_comp"
  Saturation4/1 -> Qgp_l_min_raw/1, Goto23/1, Goto61/1, Gain14/1, Gain12/1
  Constant11/1 -> Product14/2, Product15/2
  [y_kalman] -> Unit Delay3/1
  Unit Delay14/1 -> MATLAB Function2/14(Ugp)
  [Delta_P1_P2_Pa] -> Gain9/1  "pascal"
  Rk_Gain_P1/1 -> Mux4/1
  Gain39/1 -> [Qvad_kalman], Qvad_l_min_kalman1/1
  Saturation5/1 -> [Air_Tank_Fill_Current]
  Demux2/1 -> [P1_Pa]
  ADC_CLASS1_BL2/1 -> Bar2Pa1/1  "Analog Ch 2"
  Gain15/1 -> P1ref/1
  [gp_PWM] -> Unit Delay14/1
  Demux1/1 -> [E1]
  Divide4/1 -> m3/sec to l/min3/1
  Saturation/1 -> g1/1, [g1]
  P1/1 -> Mux2/1
  Gain7/1 -> P2_p_mmHg_raw/1, [P2p_mmHg_raw]
  Gain40/1 -> Scope2/1, Saturation18/1
  [E3] -> P3 Fill/1(error)
  [P2p_Pa_raw] -> P2_p/1
  Constant4/1 -> P2 Fill/4(difference)
  Demux2/4 -> [P3_Pa]
  Saturation6/1 -> [Ao_Fill_current]
  [E2] -> P2 Fill/1(error)
  Qk_Gain_Qgp/1 -> Mux/6
  Gain/1 -> [P3_mmHg_raw], Pin_mmHg_raw/1, P3_mmHg_raw/1, [Pin_mmHg_raw]
  [Delta_P3_Patm_Pa] -> Divide4/2
  Constant5/1 -> P2 Release/4(difference)
  Demux/5 -> Saturation13/1
  ADC_CLASS1_BL13/1 -> Gain13/1  "Flow Sensor 2"
  Demux/1 -> Saturation/1
  PWM Period1/1 -> DIO_CLASS1_PWM_BL3/1
  Add3/1 -> [Delta_P3_Patm_Pa], Delta_P2_tank_atm_Pa2/1  "pascal"
  [Q_PLV_Release] -> P3 Release/3(Q_Calculated)
  [P_kalman] -> Unit Delay5/1
  [y_kalman] -> Unit Delay10/1
  Gain20/1 -> [P2_mmHg], P2_mmHg_kalman/1, Pout_mmHg_kalman/1, [Pout_mmHg]
  Gain26/1 -> Pvac_mmHg/1
  [Q_P1_Tank_Fill] -> Compressor to P1 Fill/3(Q_Calculated)
  MATLAB Function2/2(P_kalman_out) -> "Pkalman "/1, [P_kalman]
  Rk_Gain_Qvad/1 -> Mux4/7
  [P1_Pa] -> Add5/1  "pascal"
  Rk_Gain_Qgp/1 -> Mux4/6
  [Delta_P1_P3_Pa] -> Divide3/2
  Saturation3/1 -> Gain11/1, Gain6/1, Goto59/1, Qlvad_l_min_raw/1, Goto73/1
  Vacuum Bias/1 -> Bar2Pa6/1
  Gain29/1 -> P3 Release/2(Measured_Delta_P)  "MPa"
  Subtract2/1 -> DP_ref/1
  Pc/1 -> MATLAB Function2/5(Pc)
  [P_Vac_Pa] -> Add6/2
  ADC_CLASS1_BL12/1 -> Vacuum Bias/1  "Analog Ch 4"
  Qk_Gain_P3/1 -> Mux/4
  P2 Fill/1(input_Current) -> Saturation6/1
  Bar2Pa/1 -> Bias10/1  "P1_Pa"
  ADC_CLASS1_BL7/1 -> Gain4/1  "Flow Sensor 1"
  Qk_Gain_P1/1 -> Mux/1
  PVac/1 -> MATLAB Function2/7(Pvac)
  P3ref/1 -> Mux3/3
  Demux/4 -> Saturation12/1
  Switch1/1 -> Subtract2/2, [P3_ref_mmHg], Gain31/1, P3_ref_mmhg/1
  Gain19/1 -> Bar2Pa2/1
  Sum18/1 -> Saturation19/1
  Mux3/1 -> MATLAB Function2/11(ref), Unit Delay4/1
  Add2/1 -> [Delta_P1_P3_Pa], Delta_P_tank_Pa2/1  "pascal"
  Saturation9/1 -> Product7/2, Product6/2, Product2/2, Product3/2, Goto47/1
  Add15/1 -> Product/2
  D_1_Sp/1 -> Product5/1
  Bias4/1 -> Saturation4/1
  Product/1 -> Sum18/1
  K4/1 -> Mux1/4
  Gain31/1 -> Scope/2, P3ref/1
  Rk_Gain_P3p/1 -> Mux4/5
  Divide2/1 -> m3/sec to l/min1/1
  MATLAB Function8/1(y) -> sat5/1  "duty_g5"
  MATLAB Function2/3(G) -> Demux/1
  ADC_CLASS1_BL11/1 -> Bar2Pa5/1  "Analog Ch 4"
  From4/1 -> Integrator7/2
  P3_sin1/1 -> Add7/1
  Upper Limit of Q = 110/1 -> [Q_P1_Tank_Fill], Q1/1
  Saturation10/1 -> [LV_Fill_current]
  Gain11/1 -> Goto60/1, Qlvad_m3_s_raw/1
  K5/1 -> Mux1/5
  Ao_tank_fill_current/1 -> MATLAB Function4/1(u), g2_current/1  "mA"
  [Q_PLV_Fill] -> P3 Fill/3(Q_Calculated)
  Divide1/1 -> m3/sec to l/min2/1
  [Q_PAo_Release] -> P2 Release/3(Q_Calculated)
  P2ref/1 -> Mux3/2
  Bias11/1 -> P2_Pa_raw/1, [P2_Pa_raw], Gain3/1
  [Delta_P3_Patm_Pa] -> Gain29/1  "pascal"
  Gain23/1 -> P1_mmHg_kalman/1
  P2_p/1 -> Mux2/2
  sat3/1 -> Product3/1
  Gain32/1 -> [P3p_mmHg], P3p_mmHg_kalman/1
  Unit Delay4/1 -> MATLAB Function2/12(ref_pre)
  P1ref/1 -> Mux3/1
  Bias3/1 -> Saturation3/1
  Qk_Gain_P3p/1 -> Mux/5
  m3/sec to l/min2/1 -> "Upper Limit of Q = 70 _2 "/1  "Q_opt_comp"
  Gain14/1 -> Qgp_ml_min_raw/1
  Qin/1 -> MATLAB Function2/8(Qp)
  ADC_CLASS1_BL3/1 -> Gain19/1
  Demux1/3 -> [E3]
  I_1_Sp/1 -> Product4/1
  Mux2/1 -> MATLAB Function2/6(z_meas)
  Saturation13/1 -> g5/1, [g5]
  Sum17/1 -> Derivative5/1, Integrator7/1, Product8/2
  gp_on_off/1 -> Product11/1, Goto48/1
  Gain8/1 -> P2 Release/2(Measured_Delta_P)  "MPa"
  Demux1/2 -> [E2]
  Gain4/1 -> Bias3/1
  [P3p_Pa] -> Add3/1  "pascal"
  Demux2/5 -> [P3p_Pa]
  Unit Delay10/1 -> Unit Delay9/1
  Add4/1 -> Delta_P_compressor_Pa1/1, [Delta_Pc_P1_Pa]  "pascal"
  P3_sin2/1 -> Add7/2
  Compressor to P1 Fill/1(input_Current) -> Saturation5/1
  MATLAB Function2/1(y_kalman_out) -> Demux2/1, [y_kalman]
  Gain6/1 -> Qlvad_ml_min_raw/1
  [P_Vac_Pa] -> Add3/2
  [Qlvad_m3_s_raw] -> Q_vad/1
  Demux2/3 -> [P2_Pa]
  ADC_CLASS1_BL1/1 -> Bar2Pa/1  "Analog Ch 1"
  Add7/1 -> Switch1/3
  [Rk] -> MATLAB Function2/4(Rk)
  [Qout_m3_s_raw] -> Qout/1
  Saturation2/1 -> g3/1, [g3]
  [P1_Pa] -> Add4/2  "pascal"
  [Pc_Pa] -> Add4/1  "pascal"
  Qout/1 -> MATLAB Function2/9(Qs)
  [g5] -> Divide4/1
  Demux/3 -> Saturation2/1
  [P2_Pa] -> P2_Pa_kalman/1, Gain20/1
  Product5/1 -> Add15/3
  LV_release_current/1 -> g5_current/1, MATLAB Function8/1(u)  "mA"
  P2/1 -> Mux2/3
  sat2/1 -> Product2/1
  P2_sin1/1 -> Add/1
  Saturation1/1 -> [g2], g2/1
  [P3p_Pa] -> Gain32/1
  MATLAB Function7/1(y) -> Product15/1  "duty_G4"
  Demux2/7 -> [Qvad_m3_s]
  [Qgp_m3_s_raw] -> Q_gp/1
  K_1_Sp/1 -> Product8/1
  PWM Period2/1 -> DIO_CLASS1_PWM_BL1/1
  Product14/1 -> sat2/1
  CVS_on_off/1 -> Goto49/1, Switch1/2, Switch/2
  Bar2Pa6/1 -> Pvac_Pa_raw1/1, [P_Vac_Pa], Gain26/1  "Vacuum_Pa"
  [P1_Pa] -> Gain23/1
  [Qin_m3_s_raw] -> Qin/1
  Enable_pin/1 -> Product16/2, Goto74/1, DIO_CLASS1_BIT_OUT_BL1/1, Goto70/1
  LV_tank_fill_current/1 -> g4_current/1, MATLAB Function7/1(u)  "mA"
  K3/1 -> Mux1/3
  [Delta_Pc_P1_Pa] -> Gain10/1  "pascal"
  [P_Vac_Pa] -> PVac/1
  [P2_Pa_raw] -> P2/1
  MATLAB Function4/1(y) -> Product14/1  "duty_G2"
  ON_OF_SP/1 -> Product/1, Goto69/1
  Add/1 -> Switch/3
  [P3p_Pa_raw] -> P3_p/1
  Saturation11/1 -> [LV_release_input_Current]
  Bar2Pa2/1 -> Gain18/1, Pcomp_Pa_raw/1, [Pc_Pa]  "Pcomp_Pa"
  Gain10/1 -> Compressor to P1 Fill/2(Measured_Delta_P)  "MPa"
  [Pc_Pa] -> Pc/1
  Integrator7/1 -> Product4/2
  m3/sec to l/min4/1 -> Upper Limit of Q = 70 _2 1/1  "Q_opt_comp"
  PWM Period5/1 -> DIO_CLASS1_PWM_BL6/1
  [Delta_P2_Patm_Pa] -> Divide2/2
  Bar2Pa1/1 -> Bias11/1  "P2t_Pa"
  Gain30/1 -> P3_p_mmHg_raw/1, [P3p_mmHg_raw]
  P3_p/1 -> Mux2/5
  K2/1 -> Mux1/2
  Mux1/1 -> MATLAB Function2/13(K_Lya)
  PWM Period6/1 -> DIO_CLASS1_PWM_BL8/1
  Derivative5/1 -> Product5/2
  Add5/1 -> Delta_P_tank_Pa1/1, [Delta_P1_P2_Pa]  "pascal"
  SP_pwm_override/1 -> Sum18/2
  Gain9/1 -> P2 Fill/2(Measured_Delta_P)  "MPa"
  Add6/1 -> [Delta_P2_Patm_Pa], Delta_P2_tank_atm_Pa1/1  "pascal"
  [g3] -> Divide2/1
  PWM Period4/1 -> DIO_CLASS1_PWM_BL4/1
  Sum/1 -> DIO_CLASS1_PWM_BL4/2, G5_PWM/1
  Sum4/1 -> DIO_CLASS1_PWM_BL2/2, G4_PWM/1
  Sum5/1 -> G3_PWM/1, DIO_CLASS1_PWM_BL1/2
  Sum7/1 -> DIO_CLASS1_PWM_BL3/2, G2_PWM/1
  VAD_ref_Q/1 -> Sum2/1
  Motor_RPM_Override/1 -> Sum1/2
  Product13/1 -> Add21/1
  Product10/1 -> Integrator4/1
  Product12/1 -> Derivative3/1
  Sum2/1 -> Product13/2, Product10/2, Product12/2
  PVAD/1 -> Product13/1
  IVAD/1 -> Product10/1
  DVAD/1 -> Product12/1
  From67/1 -> Integrator4/2
  Sum1/1 -> DTM_RPM/1, Product16/1
  Product16/1 -> Gain40/1
  From76/1 -> Sum17/2
  gp_pwm_override/1 -> Sum3/2
  Product11/1 -> "IBS_o "/1, Sum3/1
  Sum3/1 -> Product20/1
  Motor PWM Period/1 -> DIO_CLASS1_PWM_BL7/1
  Saturation16/1 -> Motor_PWM/1, DIO_CLASS1_PWM_BL7/2
  Fcn/1 -> Switch2/1
  Switch2/1 -> Saturation16/1
  Constant/1 -> Switch2/3
  Gain2/1 -> Bias1/1
  ADC_CLASS1_BL8/1 -> Gain2/1  "Flow Sensor 1"
  Bias1/1 -> Saturation20/1
  From74/1 -> Add10/1
  From73/1 -> Add10/2
  Add10/1 -> Gain35/1, Goto22/1, LVAD_BS/1
  Gain25/1 -> Transfer Fcn1/1
  Gain27/1 -> Transfer Fcn/1
  Transfer Fcn/1 -> [Q_LA_Ref]
  Transfer Fcn1/1 -> [Q_LV_Ref]
  Gain35/1 -> Goto12/1
  Small_Pump_Ref/1 -> "ref_sp "/1, Sum17/1
  PWM Period3/1 -> DIO_CLASS1_PWM_BL2/1
  Unit Delay/1 -> Add11/2
  Unit Delay1/1 -> Add12/1
  Gain37/1 -> Qsp_ml_min_raw/1
  Saturation20/1 -> Gain36/1, Gain37/1, Goto66/1, Qsp_l_min_raw/1
  Gain36/1 -> Goto76/1, Qsp_m3_s_raw/1
  Qk_Gain_Qvad1/1 -> Mux/8
  Qk_Gain_Qvad/1 -> Mux/7
  Rk_Gain_Qsp/1 -> Mux4/8
  Q_sp/1 -> Mux2/8
  [SP_m3_s_raw] -> Q_sp/1
  Demux2/8 -> [Qsp_m3_s]
  Gain41/1 -> Qsp_l_min_kalman/1, [Qsp_kalman]
  [Qsp_m3_s] -> Gain41/1
  Reference CVSs/4(QLA) -> Gain27/1
  Reference CVSs/3(QLV) -> Gain25/1
  Reference CVSs/2(PLV_ref) -> Unit Delay1/1
  Reference CVSs/1(PA_ref) -> Unit Delay/1
  Gain42/1 -> Motor_PWM1/1
  Motor PWM/1 -> Fcn/1, Switch2/2
  Gain22/1 -> [P2p_mmHg], P2p_mmHg_kalman/1
  KALMAN 3 STATES PLA/1(Output) -> ?
  Product20/1 -> Saturation17/1
  GP_KAPATT/1 -> Product20/2
  Saturation8/1 -> DTM_RPM1/1
  VAD_PID_ON_OFF/1 -> Product9/2
  IBS_LVAD/1(W) -> Saturation8/1
  Product9/1 -> Sum1/1
  Derivative3/1 -> Add21/3
  Integrator4/1 -> Add21/2
  From34/1 -> Sum2/2
  Bias8/1 -> P3p_Pa_raw/1, [P3p_Pa_raw], Gain30/1
  Bias9/1 -> P2p_Pa_raw/1, [P2p_Pa_raw], Gain7/1
  Bias10/1 -> P3_Pa_raw/1, [P3_Pa_raw], Gain/1
  PID_of_PID_ITM/1 -> Switch7/2, PID Controller/5
  PID_of_I/1 -> PID Controller/3
  PID_of_D/1 -> PID Controller/4
  ref_of_ITM/1 -> Sum6/1
  From35/1 -> Sum6/2
  PID Controller/1 -> Error_ITM/1, Switch7/1
  PID_of_P/1 -> PID Controller/2
  Sum6/1 -> PID Controller/1
  Constant12/1 -> PID_of_I/1, PID_of_P/1, PID_of_D/1
  ADC_CLASS1_BL14/1 -> raw_rpm/1, Relational Operator/1, Compare To Zero/1
  Relational Operator/1 -> ed_de1/1, Edge Detector1/1
  Unit Delay2/1 -> MATLAB Function9/3(tt_pre)
  MATLAB Function9/2(tt) -> Unit Delay2/1
  Edge Detector1/1 -> MATLAB Function9/1(C), edge_de/1
  Clock3/1 -> MATLAB Function9/2(t)
  Divide9/1 -> Divide8/2
  Divide8/1 -> Moving Average/1, RPM_read/1, Display1/1
  Moving Average/1 -> RPM_read2/1
  Constant21/1 -> Divide9/1
  Constant2/1 -> Relational Operator/2
  Constant20/1 -> Divide8/1
  Unit Delay6/1 -> Scope14/1, Divide9/2
  Moving Average1/1 -> Display/1, rpm_mov_per/1, Unit Delay6/1
  MATLAB Function9/1(per) -> per/1, Moving Average1/1
  Gain17/1 -> P1_mmHg_raw/1
  Bar2Pa4/1 -> Gain17/1, P1_Pa_raw/1, [P1_Pa_raw]  "Pairtank_Pa"
  ADC_CLASS1_BL5/1 -> Gain34/1  "Analog C 5"
  Gain34/1 -> Bar2Pa4/1
  Product7/1 -> Sum/1
  LV_r_ow/1 -> Sum/2
  LV_f_ow/1 -> Sum4/2
  Product6/1 -> Sum4/1
  AO_r_ow/1 -> Sum5/2
  Product3/1 -> Sum5/1
  AO_f_ow/1 -> Sum7/2
  Product2/1 -> Sum7/1
  ? -> Scope1/1
  From3/1 -> Subsystem1/1(Qvad)
  DV_calc/1(Out1) -> Subsystem1/3("DV ")
  DP_calc/1(Out1) -> Subsystem1/2(DP)
  Subsystem1/1(Out1) -> Product11/2
